simulink model "HAE"  (R2018a)
settings: Solver=ode4  StartTime=0  StopTime=2  MaxStep=1e-4  RelTol=1e-3
InitFcn:
  | close
  | clear
  | clc
  | Sc=128
  | f=60;
  | T=1/f;
  | Ts=1/(f*Sc);
  | Vr=6500
  | V_v=[1    0.4    1          0.6       1       0.6       1       0.75   0.95]
  | T_v=[0   20/f  70/f    200/f   300/f     330/f   400/f   500/f  10]
  | S_time=60/f*20.5
  | V_R=3;
  | Tf=3
  | T_lc=3
  | set_param('HAE/EMISOR-RECEPTOR/TCP_IP_RX1/ESCRITURA', 'Value','0')
  | set_param('HAE/EMISOR-RECEPTOR/TCP_IP_RX1/RETARDO', 'Value','0')
  | run script_client_1_inicio2.m
undefined symbols (not defined in the file or in its folder): D11, Delta, DiscIntNeverNeededParam, Int, Ip1
libraries: powerlib x68, simulink x12, powerlib_meascontrol x6, libreria_comunicaciones_cliente2 x2, libreria_medidores2 x1
(part 1 of 5)
settings Model: Creator=Mateo  LastModifiedBy=ana-n
settings CodeAppCC: StateflowObjectComments=on
settings SimscapeCC: SimscapeNormalizeSystem=off

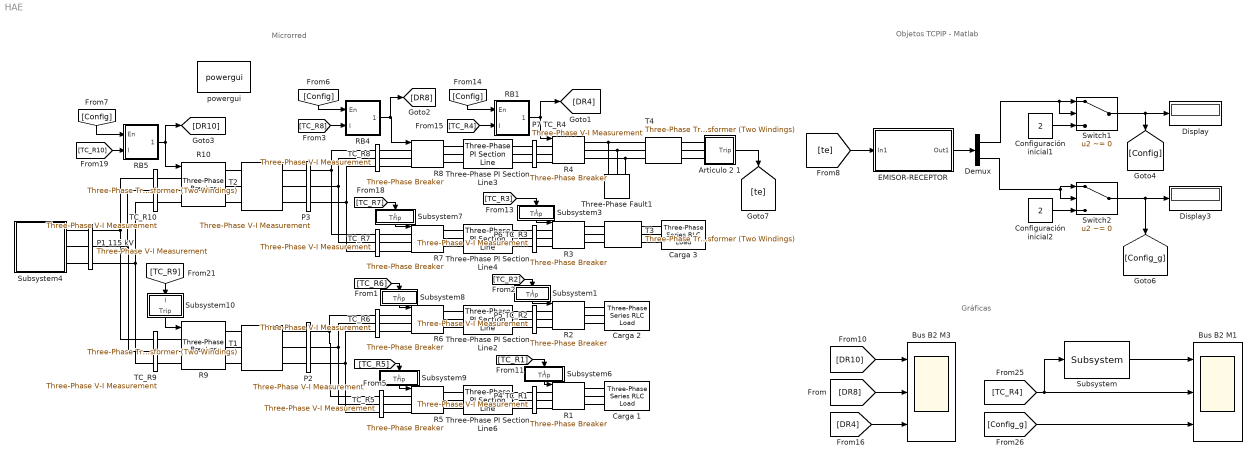
== system HAE ==
  note: Microrred
  note: Gráficas
  note: Objetos TCPIP - Matlab
  Articulo 2 1 : Subsystem  mask(Electric Arc Furnace Hyperbolic Model){Vp=200, Vat=50, m_Vat=0.01, RZs1=0.0528e-10, HZs1=1.4897e-10, RZc1=0.3366e-3, HZc1=0.01025e-3, Ci=190e3, Cd=39e3, Di_Dd=5e3, Constant_stages=[1 2 -15 0.5]}
      mask prompts: Vp "Peak Voltage"; RZs1 "RZs1 resistance Zs1"; HZs1 "HZs1 inductance Zs1"; RZc1 "RZc1 resistance Zc1"; HZc1 "HZc1 inductance Zc1"; Ci "Constant arc power Ci"; Cd "Constant arc power Cd"; Di_Dd "Constant arc current Did"; Constant_stages "Constants of each stage"
      mask help:
      | This model is based on the following documents:
      |
      | -Review on characteristic modeling of electric arc and its effects furnace
      | -Power system harmonics Computer modelling and analysis de Henrique Hacha y Manuel Madrigal
      | -Hornos de arco electrico Una vision desde la calidad de la potencia electrica
      |
      | This model recreates the time-varying, non-linear load behavior of the Electric Arc Furnaces.
      |
      | This model includes the possibility to add a time interval of different stages  of the tap-to-tap cycle as:
      |
      | -Furnance charging
      | -Melting.
      | -Refining
      | -De-slaging
      | -Furnace Turn-over
      |
      | The tap-to-tap cycle runs  through the simulation repeating the time intervals of the tap-to-tap cycle with different magnitudes in each cycle.
      |
      | The time of tap-to-tap cycle can be found in the book "Hornos de arco electrico Una vision desde la calidad de la potencia electrica" Table 2.3
      |
      | Additionaly considers the:
      | -Drilling period: Short period (between 3 to 4 minutes) using reduced voltages and powers. The material to be reduced, cause very irregular variations in the electric arc.
      | -Melting period: The electric arc is surrounded by melting scrap, which at this stage forms a more homogeneous material than in the drilling period. Full voltage and power is used in this process, lasting between 21 to 23 minutes. Typical values for medium power electric furnace are 610 V, 42 kA, 37 MW and PF 0.83.
      | -End of melting period and reheating: Uses lower voltage and higher current than in the melting period. It involves short arcs and last for about 5 minutes. Typical values in this process are 560 V, 45 kA, 34 MW and PF 0.78.
      |
      | To control the operation time of each of stages of the Tap-to-tap cycle, inside the model are differenciated as follows:
      | 1- Furnace charging
      | 2- Melting
      | 3- Refining and De-slaging
      | 4- Furnace turn-over
      mask Help:
      | This document implements the model of the Electric Arc Furnace (EAF) based on the following hyperbolic model.
      | 
      | V(I)=[V_T+(Ci,d)/(Di,d+abs(I))]signum(I)
      | 
      | Where I and V are the arc current and voltage of a given phase, respectively. In addition, V_T is the magnitude of the voltage threshold to which the voltage approaches as the current increases. This voltage is dependent on the arc length. Constants Ci,d and Di,d are corresponding to the arc power and arc current respectively, and regarding the sign of the derivative of the arc current, they can take different values. Since this equation is similar to the hyperbolic function, it is named hyperbolic model. There are different paths to increase or reduce the current.
      | 
      | The first describes the increasing current I(t), and the second the decreasing current (d).
      | 
      | Thus, constans Ci,d and Di,d are distinguised. The constants for the first path are Ci and Di and constans of the second path are Cd and Dd.
      | 
      | This model contemplates the possibility to change the time interval of the tap-to-tap cycle operation.
      | The so-called ultra-high-power furnaces, available since 1960, can have capacities of 50-150 tonnes, can have 12 melting cycles per day, opposed with 4 to 5 cycles achieved with previeous generations of furnaces.
      | 
      | Large variations are observed in the voltage and current measured during the drilling period, giving rise to a badly distorted v-i characteristic, which resembles more a transient operation than the steady-state operation. During the melting-down process the voltage and current waveforms are more regular but still the voltage is highly non-sinusoidal. At the end of the melting-down period, the voltage waveform becomes more sinusoidal and the v-i characteristic exhibits a high degree of linearity.
      | 
      | Rated Power of the transformer: 30 MVA
      | Transformer relation of the transformer 115/13.8 kV
      | Impedance of short circuit: 10,27% at 25 MVA
      | 
      | Rated short circuit power of the grid of the point of common coupling (115 kV).
      | Short circuit rated power 1653 MVA
      | Short circuit current 8300 A
      | 
      | Impedance of the transformer of the EAF. (Toshiba recommends)
      | Impedance Z% 5% - 6%
      | 
      | Maximun voltage at the secundary of the transformer.
      | Vmax=700 V
      | 
      | The time of the refining depends on the amount of tonns required (example of 38 Tonns). The EAF uses a 120 kWh/Tonn. Therefore,
      | 
      | E_required=(120kWh/Tonn)*(38 Tonn)=4560 kWh
      | 
      | - Complicated refining (more time required):
      | 
      | In consequence, the active required power is:
      | 
      | P_required=E_required/t_max_refining=4560 kWh*(60min/1h)*(1/40min)=6,8 MW
      | 
      | With the required active power is possible to compute the required aparent power (S) using the estimated power factor.
      | 
      | S_required=P_required/FP=6,8 MW/0,8 = 8,6 MVA
      | 
      | With a voltage of 380V the current is:
      | 
      | I=S_required/(sqrt(3)*V)=8,6MW/(sqrt(3)*380V)=13,1 kA
      | 
      | - Refining:
      | 
      | Refining stage: using the same EAF for the proces of refining, the estimated production takes t_max_refining = 20 min.
      | With this time the required power takes:
      | 
      | P_required=4560 kWh*(60min/1h)*(1/20min)=12,7 MW
      | S_required=12,7 MW/0,8 = 17 MVA
      | 
      | For a voltage of 500 V:
      | I=17MW/(sqrt(3)*500V)=19,6 kA
      | 
      | - Fusion stage
      | 
      | Fusion stage requires 400 kWh/T. Additionally the modeled EAF uses burners that use 466 kWh/min
      | 
      | E_required=(400kWh/Tonn)*(33 Tonn)=13200 kWh
      | t_fusion=E_required/Burning=13200 kWh/466 kWh/min=28 min
      | 
      | Wihtout burners, the Burning takes 400 kWh/min
      | 
      | t_fusion=E_required/Burning=13200 kWh/400 kWh/min=33 min
      | 
      | - Time of charging and turn-over
      | 
      | The time of the charging to transport the scrapping and how to fill the furnace. Estimating 4 loads to charge the furnace in 3 minutes it takes.
      | 
      | t_charging=(# charging)*(time of charging)=4*3 min=12 min
      | Time of turn-over: 10 minutes.
      | 
      | Therefore, consider a time interval for the tap-to-tap cycle of 60 min - 85 min, as follows:
      | 
      | -Furnace Charging: 12 minutes
      | -Melting: 28 minutes
      | -Refining and De-slaging: 20 minutes
      | -Furnace turn-over: 10 minutes
      | 
      | Considering 70 cycles as a hole tap-to-tap cycle, the following time interval is considered:
      | 
      | -Furnace Charging: 12 cycles
      | -Melting: 28 cycles
      | -Refining and De-slaging: 20 cycles
      | -Furnace turn-over: 10 cycles
      mask Display: disp('HAE');
  Bus B2 M1 : Scope  NumInputPorts=3
  Bus B2 M3 : Scope  NumInputPorts=3
  Carga 1 : powerlib/Elements/Three-Phase Series RLC Load  LConnTagsString=A|B|C  Configuration=Y (grounded)  NominalVoltage=13.8e3  Vabc=[1e3 1e3 1e3]  Vabcp=[1e3 1e3 1e3]  NominalFrequency=60  UnbalancedPower=off  ActivePower=35e5  InductivePower=3e5  CapacitivePower=0  Pabc=[10e3 9e3 11e3]  QLabc=[100 90 110]  QCabc=[100 90 110]  Pabcp=[10e3 9e3 11e3]  QLabcp=[100 90 110]  QCabcp=[100 90 110]  Measurements=None  LoadType=constant PQ
  Carga 2 : powerlib/Elements/Three-Phase Series RLC Load  LConnTagsString=A|B|C  Configuration=Y (grounded)  NominalVoltage=13.8e3  Vabc=[1e3 1e3 1e3]  Vabcp=[1e3 1e3 1e3]  NominalFrequency=60  UnbalancedPower=off  ActivePower=35e5  InductivePower=3e5  CapacitivePower=0  Pabc=[10e3 9e3 11e3]  QLabc=[100 90 110]  QCabc=[100 90 110]  Pabcp=[10e3 9e3 11e3]  QLabcp=[100 90 110]  QCabcp=[100 90 110]  Measurements=None  LoadType=constant PQ
  Carga 3 : powerlib/Elements/Three-Phase Series RLC Load  LConnTagsString=A|B|C  Configuration=Y (grounded)  NominalVoltage=0.480e3  Vabc=[1e3 1e3 1e3]  Vabcp=[1e3 1e3 1e3]  NominalFrequency=60  UnbalancedPower=off  ActivePower=6e6  InductivePower=0.5e6  CapacitivePower=0  Pabc=[10e3 9e3 11e3]  QLabc=[100 90 110]  QCabc=[100 90 110]  Pabcp=[10e3 9e3 11e3]  QLabcp=[100 90 110]  QCabcp=[100 90 110]  Measurements=None  LoadType=constant PQ
  Configuración inicial1 : Constant  Value=2
  Configuración inicial2 : Constant  Value=2
  Demux : Demux  Outputs=2
  Display : Display
  Display3 : Display
  EMISOR-RECEPTOR : Subsystem
      mask Display: disp("Emisor-Receptor")
  P1 115 kV : powerlib/Measurements/Three-Phase V-I Measurement  VoltageMeasurement=phase-to-ground  SetLabelV=on  LabelV=V_B_P1  Vpu=off  VpuLL=off  CurrentMeasurement=yes  SetLabelI=on  LabelI=I_B_P1  Ipu=off  Pbase=100e6  Vbase=500e3  OutputType=Complex  PhasorSimulation=off  PSBequivalent=0
  P2 : powerlib/Measurements/Three-Phase V-I Measurement  VoltageMeasurement=phase-to-ground  SetLabelV=on  LabelV=V_F_F2  Vpu=off  VpuLL=off  CurrentMeasurement=yes  SetLabelI=on  LabelI=I_F_F2  Ipu=off  Pbase=100e6  Vbase=500e3  OutputType=Complex  PhasorSimulation=off  PSBequivalent=0
  P3 : powerlib/Measurements/Three-Phase V-I Measurement  VoltageMeasurement=phase-to-ground  SetLabelV=on  LabelV=V_F_F3  Vpu=off  VpuLL=off  CurrentMeasurement=yes  SetLabelI=on  LabelI=I_F_F3  Ipu=off  Pbase=100e6  Vbase=500e3  OutputType=Complex  PhasorSimulation=off  PSBequivalent=0
  P4 TC_R1 : powerlib/Measurements/Three-Phase V-I Measurement  VoltageMeasurement=phase-to-ground  SetLabelV=on  LabelV=V_RM_1  Vpu=off  VpuLL=off  CurrentMeasurement=yes  SetLabelI=on  LabelI=TC_R1  Ipu=off  Pbase=100e6  Vbase=500e3  OutputType=Complex  PhasorSimulation=off  PSBequivalent=0
  P5 TC_R2 : powerlib/Measurements/Three-Phase V-I Measurement  VoltageMeasurement=phase-to-ground  SetLabelV=on  LabelV=V_F_RM_2  Vpu=off  VpuLL=off  CurrentMeasurement=yes  SetLabelI=on  LabelI=TC_R2  Ipu=off  Pbase=100e6  Vbase=500e3  OutputType=Complex  PhasorSimulation=off  PSBequivalent=0
  P6 TC_R3 : powerlib/Measurements/Three-Phase V-I Measurement  VoltageMeasurement=phase-to-ground  SetLabelV=on  LabelV=V_HV_L3  Vpu=off  VpuLL=off  CurrentMeasurement=yes  SetLabelI=on  LabelI=TC_R3  Ipu=off  Pbase=100e6  Vbase=500e3  OutputType=Complex  PhasorSimulation=off  PSBequivalent=0
  P7 TC_R4 : powerlib/Measurements/Three-Phase V-I Measurement  VoltageMeasurement=phase-to-ground  SetLabelV=on  LabelV=V_HV_7  Vpu=off  VpuLL=off  CurrentMeasurement=yes  SetLabelI=on  LabelI=TC_R4  Ipu=off  Pbase=100e6  Vbase=500e3  OutputType=Complex  PhasorSimulation=off  PSBequivalent=0
  R1 : powerlib/Elements/Three-Phase Breaker  InitialState=closed  SwitchA=on  SwitchB=on  SwitchC=on  SwitchTimes=[5]  External=on  BreakerResistance=0.001  SnubberResistance=1e6  SnubberCapacitance=inf  Measurements=None
      link override Breaker A: Measurements=None
      link override Breaker B: Measurements=None
      link override Breaker C: Measurements=None
  R10 : powerlib/Elements/Three-Phase Breaker  InitialState=closed  SwitchA=on  SwitchB=on  SwitchC=on  SwitchTimes=[5]  External=on  BreakerResistance=0.001  SnubberResistance=1e6  SnubberCapacitance=inf  Measurements=None
      link override Breaker A: Measurements=None
      link override Breaker B: Measurements=None
      link override Breaker C: Measurements=None
  R2 : powerlib/Elements/Three-Phase Breaker  InitialState=closed  SwitchA=on  SwitchB=on  SwitchC=on  SwitchTimes=[5]  External=on  BreakerResistance=0.001  SnubberResistance=1e6  SnubberCapacitance=inf  Measurements=None
      link override Breaker A: Measurements=None
      link override Breaker B: Measurements=None
      link override Breaker C: Measurements=None
  R3 : powerlib/Elements/Three-Phase Breaker  InitialState=closed  SwitchA=on  SwitchB=on  SwitchC=on  SwitchTimes=[5]  External=on  BreakerResistance=0.001  SnubberResistance=1e6  SnubberCapacitance=inf  Measurements=None
      link override Breaker A: Measurements=None
      link override Breaker B: Measurements=None
      link override Breaker C: Measurements=None
  R4 : powerlib/Elements/Three-Phase Breaker  InitialState=closed  SwitchA=on  SwitchB=on  SwitchC=on  SwitchTimes=[20]  External=on  BreakerResistance=0.001  SnubberResistance=1e6  SnubberCapacitance=inf  Measurements=None
      link override Breaker A: Measurements=None
      link override Breaker B: Measurements=None
      link override Breaker C: Measurements=None
  R5 : powerlib/Elements/Three-Phase Breaker  InitialState=closed  SwitchA=on  SwitchB=on  SwitchC=on  SwitchTimes=[5]  External=on  BreakerResistance=0.001  SnubberResistance=1e6  SnubberCapacitance=inf  Measurements=None
      link override Breaker A: Measurements=None
      link override Breaker B: Measurements=None
      link override Breaker C: Measurements=None
  R6 : powerlib/Elements/Three-Phase Breaker  InitialState=closed  SwitchA=on  SwitchB=on  SwitchC=on  SwitchTimes=[5]  External=on  BreakerResistance=0.001  SnubberResistance=1e6  SnubberCapacitance=inf  Measurements=None
      link override Breaker A: Measurements=None
      link override Breaker B: Measurements=None
      link override Breaker C: Measurements=None
  R7 : powerlib/Elements/Three-Phase Breaker  InitialState=closed  SwitchA=on  SwitchB=on  SwitchC=on  SwitchTimes=[5]  External=on  BreakerResistance=0.001  SnubberResistance=1e6  SnubberCapacitance=inf  Measurements=None
      link override Breaker A: Measurements=None
      link override Breaker B: Measurements=None
      link override Breaker C: Measurements=None
  R8 : powerlib/Elements/Three-Phase Breaker  InitialState=closed  SwitchA=on  SwitchB=on  SwitchC=on  SwitchTimes=[20]  External=on  BreakerResistance=0.001  SnubberResistance=1e6  SnubberCapacitance=inf  Measurements=None
      link override Breaker A: Measurements=None
      link override Breaker B: Measurements=None
      link override Breaker C: Measurements=None
  R9 : powerlib/Elements/Three-Phase Breaker  InitialState=closed  SwitchA=on  SwitchB=on  SwitchC=on  SwitchTimes=[5]  External=on  BreakerResistance=0.001  SnubberResistance=1e6  SnubberCapacitance=inf  Measurements=None
      link override Breaker A: Measurements=None
      link override Breaker B: Measurements=None
      link override Breaker C: Measurements=None
  RB1 : Subsystem  mask(Proteccion de Sobrecorriente multitopologia){menu=3, TCpopup1=IEC Standard Inverse, k1=0.14, alpha1=0.02, B1=0, PS1=0.10, TMS1=0.5, Tins1=0.015, Esc1=10, TCpopup2=IEC Standard Inverse, k2=0.14, alpha2=0.02, B2=0, PS2=1, TMS2=0.060, Tins2=0.09, Esc2=5, TCpopup3=IEC Standard Inverse, k3=0.14, alpha3=0.02, B3=0, PS3=0.6267, TMS3=0.100, Tins3=0.05, Esc3=4, Vp=1200, Vs=5, F=60}
      mask prompts: menu "Numero de Topologias"; TCpopup1 "Caracteristica de Disparo"; k1 "k"; alpha1 "alpha"; B1 "B"; PS1 "Seteo disparo(PS)/Seteo inferior(I>)"; TMS1 "Multiplicador de Tiempo"; Tins1 "Tins"; Esc1 "Escala"; TCpopup2 "Caracteristica de Disparo"; k2 "k"; alpha2 "alpha"; B2 "B"; PS2 "Seteo disparo(PS)/Seteo inferior(I>)"; TMS2 "Multiplicador de tiempo"; Tins2 "Tins"; Esc2 "Escala"; TCpopup3 "Caracteristica de Disparo"; k3 "k"; alpha3 "alpha"; B3 "B"; PS3 "Seteo disparo(PS)/Seteo inferior(I>)"; TMS3 "Multiplicador de Tiempo"; Tins3 "Tins"; Esc3 "Escala"; Vp "Primario CT"; Vs "Secundario CT"; F "Frecuencia"
      mask help: Proteccion de Sobrecorriente con tres topologias internas controladas por una señal de control externa.
      mask init:
      | warning('off','Simulink:Masking:Invalid_Visible_Flag')
      mask TypeOptions menu: 1 | 2 | 3
      mask Callback menu:
      | h = getSimulinkBlockHandle(gcb);
      | menu1 = get_param(h,'menu');
      | if strcmp(menu1,num2str(1))
      |     set_param(h,'MaskVisibilities',{'on',...
      |         'on','on','on','on','on','on','on','on',...%proteccion 1 activa
      |         'off','off','off','off','off','off','off','off',...%proteccion 2 desactivada
      |         'off','off','off','off','off','off','off','off',...%proteccion 3 desactivada
      |         'on','on','on'});%Otros parametros activados
      |     Int=1;
      | elseif strcmp(menu1,num2str(2))
      |  set_param(h,'MaskVisibilities',{'on',...
      |         'on','on','on','on','on','on','on','on',...%proteccion 1 activa
      |         'on','on','on','on','on','on','on','on',...%proteccion 2 activa
      |         'off','off','off','off','off','off','off','off',...%proteccion 3 desactivada
      |         'on','on','on'});%Otros parametros activados
      |     Int=2;
      | else
      | set_param(h,'MaskVisibilities',{'on',...
      |         'on','on','on','on','on','on','on','on',...%proteccion 1 activa
      |         'on','on','on','on','on','on','on','on',...%proteccion 2 activa
      |         'on','on','on','on','on','on','on','on',...%proteccion 3 desactivada
      |         'on','on','on'});%Otros parametros activados
      |     Int=3;
      | end
      mask TypeOptions TCpopup1: IEC Standard Inverse | IEC Very Inverse | IEC Long Time Inverse | IEC Extremely Inverse | IEC Ultra Inverse | IEEE Moderately Inverse | IEEE Very Inverse | IEEE Extremely Inverse
      mask Callback TCpopup1:
      | switch(get_param(gcb,'TCpopup1'))
      |     case 'IEC Standard Inverse'
      |         set_param(gcb,'k1','0.14');
      |         set_param(gcb,'alpha1','0.02');
      |         set_param(gcb,'B1','0');
      |     case 'IEC Very Inverse'
      |         set_param(gcb,'k1','13.5');
      |         set_param(gcb,'alpha1','1');
      |         set_param(gcb,'B1','0');
      |     case 'IEC Long Time Inverse'
      |         set_param(gcb,'k1','120');
      |         set_param(gcb,'alpha1','1');
      |         set_param(gcb,'B1','0');
      |     case 'IEC Extremely Inverse'
      |         set_param(gcb,'k1','80');
      |         set_param(gcb,'alpha1','2');
      |         set_param(gcb,'B1','0');
      |     case 'IEC Ultra Inverse'
      |         set_param(gcb,'k1','315.2');
      |         set_param(gcb,'alpha1','2.5');
      |         set_param(gcb,'B1','0');
      |     case 'IEEE Moderately Inverse'
      |         set_param(gcb,'k1','0.0515');
      |         set_param(gcb,'alpha1','0.02');
      |         set_param(gcb,'B1','0.114');
      |     case 'IEEE Very Inverse'
      |         set_param(gcb,'k1','19.61');
      |         set_param(gcb,'alpha1','2');
      |         set_param(gcb,'B1','0.491');
      |     case 'IEEE Extremely Inverse'
      |         set_param(gcb,'k1','28.2');
      |         set_param(gcb,'alpha1','2');
      |         set_param(gcb,'B1','0.1217');
      | end
      | % Plotting IDMT Curve
      | clf('reset')
      | TMS = str2num(get_param(gcb,'TMS1'));
      | Vp = str2num(get_param(gcb,'Vp'));
      | PS=str2num(get_param(gcb,'PS1'));
      | k = str2num(get_param(gcb,'k1'));
      | alpha = str2num(get_param(gcb,'alpha1'));
      | B = str2num(get_param(gcb,'B1'));
      | Esc = str2num(get_param(gcb,'Esc1'));
      | Tins = str2num(get_param(gcb,'Tins1'));
      | I = [1.1:0.1:Esc];
      | I1=[Esc,Esc:0.1:30];
      | y=((k./((I.^alpha)-1))+B)*TMS;
      | Tin=[((k./((Esc.^alpha)-1))+B)*TMS,ones(1,length(I1)-1)*Tins];
      | loglog(I,y,'b');
      | hold on
      | loglog(I1,Tin,'b');
      | set(gcf, 'Position', [200 150 300 500]);
      | switch(get_param(gcb,'TCpopup1'))
      |     case 'IEC Standard Inverse'
      |         title('IEC Standard Inverse');
      |     case 'IEC Very Inverse'
      |         title('IEC Very Inverse');
      |     case 'IEC Long Time Inverse'
      |         title('IEC Long Time Inverse');
      |     case 'IEC Extremely Inverse'
      |         title('IEC Extremely Inverse');
      |      case 'IEC Ultra Inverse'
      |         title('IEC Ultra Inverse');
      |     case 'IEEE Moderately Inverse'
      |         title('IEEE Moderately Inverse');
      |     case 'IEEE Very Inverse'
      |         title('IEEE Very Inverse');
      |     case 'IEEE Extremely Inverse'
      |         title('IEEE Extremely Inverse');
      | end
      | ymax=10^ceil(log10(max(y)));
      | set(gca, 'XTick',[1:10 20]);
      | set(gca, 'YTick',[0 ymax/1000 ymax/500 ymax/200 ymax/100 ymax/50 ymax/20 ymax/10 ymax/5 ymax/2 ymax]);
      | xlim([0.9 30]);
      | ylim([0.01 ymax]);
      | xlabel(['Corriente multiplicada por Ipick-up(' num2str(PS*Vp) 'A)']);
      | ylabel('Tiempo de Operacion (Seg)');
      | grid on;
      | set(gca, 'color',[0.9608 0.9608 0.937]);
      | set(gca, 'gridcolor',[0 0.6902 0.3137]);
      mask Callback PS1:
      | % Plotting IDMT Curve
      | clf('reset')
      | TMS = str2num(get_param(gcb,'TMS1'));
      | Vp = str2num(get_param(gcb,'Vp'));
      | PS=str2num(get_param(gcb,'PS1'));
      | k = str2num(get_param(gcb,'k1'));
      | alpha = str2num(get_param(gcb,'alpha1'));
      | B = str2num(get_param(gcb,'B1'));
      | Esc = str2num(get_param(gcb,'Esc1'));
      | Tins = str2num(get_param(gcb,'Tins1'));
      | I = [1.1:0.1:Esc];
      | I1=[Esc,Esc:0.1:30];
      | y=((k./((I.^alpha)-1))+B)*TMS;
      | Tin=[((k./((Esc.^alpha)-1))+B)*TMS,ones(1,length(I1)-1)*Tins];
      | loglog(I,y,'b');
      | hold on
      | loglog(I1,Tin,'b');
      | set(gcf, 'Position', [200 150 300 500]);
      | switch(get_param(gcb,'TCpopup1'))
      |     case 'IEC Standard Inverse'
      |         title('IEC Standard Inverse');
      |     case 'IEC Very Inverse'
      |         title('IEC Very Inverse');
      |     case 'IEC Long Time Inverse'
      |         title('IEC Long Time Inverse');
      |     case 'IEC Extremely Inverse'
      |         title('IEC Extremely Inverse');
      |      case 'IEC Ultra Inverse'
      |         title('IEC Ultra Inverse');
      |     case 'IEEE Moderately Inverse'
      |         title('IEEE Moderately Inverse');
      |     case 'IEEE Very Inverse'
      |         title('IEEE Very Inverse');
      |     case 'IEEE Extremely Inverse'
      |         title('IEEE Extremely Inverse');
      | end
      | ymax=10^ceil(log10(max(y)));
      | set(gca, 'XTick',[1:10 20]);
      | set(gca, 'YTick',[0 ymax/1000 ymax/500 ymax/200 ymax/100 ymax/50 ymax/20 ymax/10 ymax/5 ymax/2 ymax]);
      | xlim([0.9 30]);
      | ylim([0.01 ymax]);
      | xlabel(['Corriente multiplicada por Ipick-up(' num2str(PS*Vp) 'A)']);
      | ylabel('Tiempo de Operacion (Seg)');
      | grid on;
      | set(gca, 'color',[0.9608 0.9608 0.937]);
      | set(gca, 'gridcolor',[0 0.6902 0.3137]);
      mask Callback TMS1:
      | % Plotting IDMT Curve
      | clf('reset')
      | TMS = str2num(get_param(gcb,'TMS1'));
      | Vp = str2num(get_param(gcb,'Vp'));
      | PS=str2num(get_param(gcb,'PS1'));
      | k = str2num(get_param(gcb,'k1'));
      | alpha = str2num(get_param(gcb,'alpha1'));
      | B = str2num(get_param(gcb,'B1'));
      | Esc = str2num(get_param(gcb,'Esc1'));
      | Tins = str2num(get_param(gcb,'Tins1'));
      | I = [1.1:0.1:Esc];
      | I1=[Esc,Esc:0.1:30];
      | y=((k./((I.^alpha)-1))+B)*TMS;
      | Tin=[((k./((Esc.^alpha)-1))+B)*TMS,ones(1,length(I1)-1)*Tins];
      | loglog(I,y,'b');
      | hold on
      | loglog(I1,Tin,'b');
      | set(gcf, 'Position', [200 150 300 500]);
      | switch(get_param(gcb,'TCpopup1'))
      |     case 'IEC Standard Inverse'
      |         title('IEC Standard Inverse');
      |     case 'IEC Very Inverse'
      |         title('IEC Very Inverse');
      |     case 'IEC Long Time Inverse'
      |         title('IEC Long Time Inverse');
      |     case 'IEC Extremely Inverse'
      |         title('IEC Extremely Inverse');
      |      case 'IEC Ultra Inverse'
      |         title('IEC Ultra Inverse');
      |     case 'IEEE Moderately Inverse'
      |         title('IEEE Moderately Inverse');
      |     case 'IEEE Very Inverse'
      |         title('IEEE Very Inverse');
      |     case 'IEEE Extremely Inverse'
      |         title('IEEE Extremely Inverse');
      | end
      | ymax=10^ceil(log10(max(y)));
      | set(gca, 'XTick',[1:10 20]);
      | set(gca, 'YTick',[0 ymax/1000 ymax/500 ymax/200 ymax/100 ymax/50 ymax/20 ymax/10 ymax/5 ymax/2 ymax]);
      | xlim([0.9 30]);
      | ylim([0.01 ymax]);
      | xlabel(['Corriente multiplicada por Ipick-up(' num2str(PS*Vp) 'A)']);
      | ylabel('Tiempo de Operacion (Seg)');
      | grid on;
      | set(gca, 'color',[0.9608 0.9608 0.937]);
      | set(gca, 'gridcolor',[0 0.6902 0.3137]);
      mask Callback Tins1:
      | % Plotting IDMT Curve
      | clf('reset')
      | TMS = str2num(get_param(gcb,'TMS1'));
      | Vp = str2num(get_param(gcb,'Vp'));
      | PS=str2num(get_param(gcb,'PS1'));
      | k = str2num(get_param(gcb,'k1'));
      | alpha = str2num(get_param(gcb,'alpha1'));
      | B = str2num(get_param(gcb,'B1'));
      | Esc = str2num(get_param(gcb,'Esc1'));
      | Tins = str2num(get_param(gcb,'Tins1'));
      | I = [1.1:0.1:Esc];
      | I1=[Esc,Esc:0.1:30];
      | y=((k./((I.^alpha)-1))+B)*TMS;
      | Tin=[((k./((Esc.^alpha)-1))+B)*TMS,ones(1,length(I1)-1)*Tins];
      | loglog(I,y,'b');
      | hold on
      | loglog(I1,Tin,'b');
      | set(gcf, 'Position', [200 150 300 500]);
      | switch(get_param(gcb,'TCpopup1'))
      |     case 'IEC Standard Inverse'
      |         title('IEC Standard Inverse');
      |     case 'IEC Very Inverse'
      |         title('IEC Very Inverse');
      |     case 'IEC Long Time Inverse'
      |         title('IEC Long Time Inverse');
      |     case 'IEC Extremely Inverse'
      |         title('IEC Extremely Inverse');
      |      case 'IEC Ultra Inverse'
      |         title('IEC Ultra Inverse');
      |     case 'IEEE Moderately Inverse'
      |         title('IEEE Moderately Inverse');
      |     case 'IEEE Very Inverse'
      |         title('IEEE Very Inverse');
      |     case 'IEEE Extremely Inverse'
      |         title('IEEE Extremely Inverse');
      | end
      | ymax=10^ceil(log10(max(y)));
      | set(gca, 'XTick',[1:10 20]);
      | set(gca, 'YTick',[0 ymax/1000 ymax/500 ymax/200 ymax/100 ymax/50 ymax/20 ymax/10 ymax/5 ymax/2 ymax]);
      | xlim([0.9 30]);
      | ylim([0.01 ymax]);
      | xlabel(['Corriente multiplicada por Ipick-up(' num2str(PS*Vp) 'A)']);
      | ylabel('Tiempo de Operacion (Seg)');
      | grid on;
      | set(gca, 'color',[0.9608 0.9608 0.937]);
      | set(gca, 'gridcolor',[0 0.6902 0.3137]);
      mask Callback Esc1:
      | % Plotting IDMT Curve
      | clf('reset')
      | TMS = str2num(get_param(gcb,'TMS1'));
      | Vp = str2num(get_param(gcb,'Vp'));
      | PS=str2num(get_param(gcb,'PS1'));
      | k = str2num(get_param(gcb,'k1'));
      | alpha = str2num(get_param(gcb,'alpha1'));
      | B = str2num(get_param(gcb,'B1'));
      | Esc = str2num(get_param(gcb,'Esc1'));
      | Tins = str2num(get_param(gcb,'Tins1'));
      | I = [1.1:0.1:Esc];
      | I1=[Esc,Esc:0.1:30];
      | y=((k./((I.^alpha)-1))+B)*TMS;
      | Tin=[((k./((Esc.^alpha)-1))+B)*TMS,ones(1,length(I1)-1)*Tins];
      | loglog(I,y,'b');
      | hold on
      | loglog(I1,Tin,'b');
      | set(gcf, 'Position', [200 150 300 500]);
      | switch(get_param(gcb,'TCpopup1'))
      |     case 'IEC Standard Inverse'
      |         title('IEC Standard Inverse');
      |     case 'IEC Very Inverse'
      |         title('IEC Very Inverse');
      |     case 'IEC Long Time Inverse'
      |         title('IEC Long Time Inverse');
      |     case 'IEC Extremely Inverse'
      |         title('IEC Extremely Inverse');
      |      case 'IEC Ultra Inverse'
      |         title('IEC Ultra Inverse');
      |     case 'IEEE Moderately Inverse'
      |         title('IEEE Moderately Inverse');
      |     case 'IEEE Very Inverse'
      |         title('IEEE Very Inverse');
      |     case 'IEEE Extremely Inverse'
      |         title('IEEE Extremely Inverse');
      | end
      | ymax=10^ceil(log10(max(y)));
      | set(gca, 'XTick',[1:10 20]);
      | set(gca, 'YTick',[0 ymax/1000 ymax/500 ymax/200 ymax/100 ymax/50 ymax/20 ymax/10 ymax/5 ymax/2 ymax]);
      | xlim([0.9 30]);
      | ylim([0.01 ymax]);
      | xlabel(['Corriente multiplicada por Ipick-up(' num2str(PS*Vp) 'A)']);
      | ylabel('Tiempo de Operacion (Seg)');
      | grid on;
      | set(gca, 'color',[0.9608 0.9608 0.937]);
      | set(gca, 'gridcolor',[0 0.6902 0.3137]);
      mask TypeOptions TCpopup2: IEC Standard Inverse | IEC Very Inverse | IEC Long Time Inverse | IEC Extremely Inverse | IEC Ultra Inverse | IEEE Moderately Inverse | IEEE Very Inverse | IEEE Extremely Inverse
      mask Callback TCpopup2:
      | switch(get_param(gcb,'TCpopup2'))
      |     case 'IEC Standard Inverse'
      |         set_param(gcb,'k2','0.14');
      |         set_param(gcb,'alpha2','0.02');
      |         set_param(gcb,'B2','0');
      |     case 'IEC Very Inverse'
      |         set_param(gcb,'k2','13.5');
      |         set_param(gcb,'alpha2','1');
      |         set_param(gcb,'B2','0');
      |     case 'IEC Long Time Inverse'
      |         set_param(gcb,'k2','120');
      |         set_param(gcb,'alpha2','1');
      |         set_param(gcb,'B2','0');
      |     case 'IEC Extremely Inverse'
      |         set_param(gcb,'k2','80');
      |         set_param(gcb,'alpha2','2');
      |         set_param(gcb,'B2','0');
      |     case 'IEC Ultra Inverse'
      |         set_param(gcb,'k2','315.2');
      |         set_param(gcb,'alpha2','2.5');
      |         set_param(gcb,'B2','0');
      |     case 'IEEE Moderately Inverse'
      |         set_param(gcb,'k2','0.0515');
      |         set_param(gcb,'alpha2','0.02');
      |         set_param(gcb,'B2','0.114');
      |     case 'IEEE Very Inverse'
      |         set_param(gcb,'k2','19.61');
      |         set_param(gcb,'alpha2','2');
      |         set_param(gcb,'B2','0.491');
      |     case 'IEEE Extremely Inverse'
      |         set_param(gcb,'k2','28.2');
      |         set_param(gcb,'alpha2','2');
      |         set_param(gcb,'B2','0.1217');
      | end
      | % Plotting IDMT Curve
      | clf('reset')
      | TMS = str2num(get_param(gcb,'TMS2'));
      | Vp = str2num(get_param(gcb,'Vp'));
      | PS=str2num(get_param(gcb,'PS2'));
      | k = str2num(get_param(gcb,'k2'));
      | alpha = str2num(get_param(gcb,'alpha2'));
      | B = str2num(get_param(gcb,'B2'));
      | Esc = str2num(get_param(gcb,'Esc2'));
      | Tins = str2num(get_param(gcb,'Tins2'));
      | I = [1.1:0.1:Esc];
      | I1=[Esc,Esc:0.1:30];
      | y=((k./((I.^alpha)-1))+B)*TMS;
      | Tin=[((k./((Esc.^alpha)-1))+B)*TMS,ones(1,length(I1)-1)*Tins];
      | loglog(I,y,'r');
      | hold on
      | loglog(I1,Tin,'r');
      | set(gcf, 'Position', [200 150 300 500]);
      | switch(get_param(gcb,'TCpopup2'))
      |     case 'IEC Standard Inverse'
      |         title('IEC Standard Inverse');
      |     case 'IEC Very Inverse'
      |         title('IEC Very Inverse');
      |     case 'IEC Long Time Inverse'
      |         title('IEC Long Time Inverse');
      |     case 'IEC Extremely Inverse'
      |         title('IEC Extremely Inverse');
      |      case 'IEC Ultra Inverse'
      |         title('IEC Ultra Inverse');
      |     case 'IEEE Moderately Inverse'
      |         title('IEEE Moderately Inverse');
      |     case 'IEEE Very Inverse'
      |         title('IEEE Very Inverse');
      |     case 'IEEE Extremely Inverse'
      |         title('IEEE Extremely Inverse');
      | end
      | ymax=10^ceil(log10(max(y)));
      | set(gca, 'XTick',[1:10 20]);
      | set(gca, 'YTick',[0 ymax/1000 ymax/500 ymax/200 ymax/100 ymax/50 ymax/20 ymax/10 ymax/5 ymax/2 ymax]);
      | xlim([0.9 30]);
      | ylim([0.01 ymax]);
      | xlabel(['Corriente multiplicada por Ipick-up(' num2str(PS*Vp) 'A)']);
      | ylabel('Tiempo de Operacion (Seg)');
      | grid on;
      | set(gca, 'color',[0.9608 0.9608 0.937]);
      | set(gca, 'gridcolor',[0 0.6902 0.3137]);
      mask Callback PS2:
      | % Plotting IDMT Curve
      | clf('reset')
      | TMS = str2num(get_param(gcb,'TMS2'));
      | Vp = str2num(get_param(gcb,'Vp'));
      | PS=str2num(get_param(gcb,'PS2'));
      | k = str2num(get_param(gcb,'k2'));
      | alpha = str2num(get_param(gcb,'alpha2'));
      | B = str2num(get_param(gcb,'B2'));
      | Esc = str2num(get_param(gcb,'Esc2'));
      | Tins = str2num(get_param(gcb,'Tins2'));
      | I = [1.1:0.1:Esc];
      | I1=[Esc,Esc:0.1:30];
      | y=((k./((I.^alpha)-1))+B)*TMS;
      | Tin=[((k./((Esc.^alpha)-1))+B)*TMS,ones(1,length(I1)-1)*Tins];
      | loglog(I,y,'r');
      | hold on
      | loglog(I1,Tin,'r');
      | set(gcf, 'Position', [200 150 300 500]);
      | switch(get_param(gcb,'TCpopup2'))
      |     case 'IEC Standard Inverse'
      |         title('IEC Standard Inverse');
      |     case 'IEC Very Inverse'
      |         title('IEC Very Inverse');
      |     case 'IEC Long Time Inverse'
      |         title('IEC Long Time Inverse');
      |     case 'IEC Extremely Inverse'
      |         title('IEC Extremely Inverse');
      |      case 'IEC Ultra Inverse'
      |         title('IEC Ultra Inverse');
      |     case 'IEEE Moderately Inverse'
      |         title('IEEE Moderately Inverse');
      |     case 'IEEE Very Inverse'
      |         title('IEEE Very Inverse');
      |     case 'IEEE Extremely Inverse'
      |         title('IEEE Extremely Inverse');
      | end
      | ymax=10^ceil(log10(max(y)));
      | set(gca, 'XTick',[1:10 20]);
      | set(gca, 'YTick',[0 ymax/1000 ymax/500 ymax/200 ymax/100 ymax/50 ymax/20 ymax/10 ymax/5 ymax/2 ymax]);
      | xlim([0.9 30]);
      | ylim([0.01 ymax]);
      | xlabel(['Corriente multiplicada por Ipick-up(' num2str(PS*Vp) 'A)']);
      | ylabel('Tiempo de Operacion (Seg)');
      | grid on;
      | set(gca, 'color',[0.9608 0.9608 0.937]);
      | set(gca, 'gridcolor',[0 0.6902 0.3137]);
      mask Callback TMS2:
      | % Plotting IDMT Curve
      | clf('reset')
      | TMS = str2num(get_param(gcb,'TMS2'));
      | Vp = str2num(get_param(gcb,'Vp'));
      | PS=str2num(get_param(gcb,'PS2'));
      | k = str2num(get_param(gcb,'k2'));
      | alpha = str2num(get_param(gcb,'alpha2'));
      | B = str2num(get_param(gcb,'B2'));
      | Esc = str2num(get_param(gcb,'Esc2'));
      | Tins = str2num(get_param(gcb,'Tins2'));
      | I = [1.1:0.1:Esc];
      | I1=[Esc,Esc:0.1:30];
      | y=((k./((I.^alpha)-1))+B)*TMS;
      | Tin=[((k./((Esc.^alpha)-1))+B)*TMS,ones(1,length(I1)-1)*Tins];
      | loglog(I,y,'r');
      | hold on
      | loglog(I1,Tin,'r');
      | set(gcf, 'Position', [200 150 300 500]);
      | switch(get_param(gcb,'TCpopup2'))
      |     case 'IEC Standard Inverse'
      |         title('IEC Standard Inverse');
      |     case 'IEC Very Inverse'
      |         title('IEC Very Inverse');
      |     case 'IEC Long Time Inverse'
      |         title('IEC Long Time Inverse');
      |     case 'IEC Extremely Inverse'
      |         title('IEC Extremely Inverse');
      |      case 'IEC Ultra Inverse'
      |         title('IEC Ultra Inverse');
      |     case 'IEEE Moderately Inverse'
      |         title('IEEE Moderately Inverse');
      |     case 'IEEE Very Inverse'
      |         title('IEEE Very Inverse');
      |     case 'IEEE Extremely Inverse'
      |         title('IEEE Extremely Inverse');
      | end
      | ymax=10^ceil(log10(max(y)));
      | set(gca, 'XTick',[1:10 20]);
      | set(gca, 'YTick',[0 ymax/1000 ymax/500 ymax/200 ymax/100 ymax/50 ymax/20 ymax/10 ymax/5 ymax/2 ymax]);
      | xlim([0.9 30]);
      | ylim([0.01 ymax]);
      | xlabel(['Corriente multiplicada por Ipick-up(' num2str(PS*Vp) 'A)']);
      | ylabel('Tiempo de Operacion (Seg)');
      | grid on;
      | set(gca, 'color',[0.9608 0.9608 0.937]);
      | set(gca, 'gridcolor',[0 0.6902 0.3137]);
      mask Callback Tins2:
      | % Plotting IDMT Curve
      | clf('reset')
      | TMS = str2num(get_param(gcb,'TMS2'));
      | Vp = str2num(get_param(gcb,'Vp'));
      | PS=str2num(get_param(gcb,'PS2'));
      | k = str2num(get_param(gcb,'k2'));
      | alpha = str2num(get_param(gcb,'alpha2'));
      | B = str2num(get_param(gcb,'B2'));
      | Esc = str2num(get_param(gcb,'Esc2'));
      | Tins = str2num(get_param(gcb,'Tins2'));
      | I = [1.1:0.1:Esc];
      | I1=[Esc,Esc:0.1:30];
      | y=((k./((I.^alpha)-1))+B)*TMS;
      | Tin=[((k./((Esc.^alpha)-1))+B)*TMS,ones(1,length(I1)-1)*Tins];
      | loglog(I,y,'r');
      | hold on
      | loglog(I1,Tin,'r');
      | set(gcf, 'Position', [200 150 300 500]);
      | switch(get_param(gcb,'TCpopup2'))
      |     case 'IEC Standard Inverse'
      |         title('IEC Standard Inverse');
      |     case 'IEC Very Inverse'
      |         title('IEC Very Inverse');
      |     case 'IEC Long Time Inverse'
      |         title('IEC Long Time Inverse');
      |     case 'IEC Extremely Inverse'
      |         title('IEC Extremely Inverse');
      |      case 'IEC Ultra Inverse'
      |         title('IEC Ultra Inverse');
      |     case 'IEEE Moderately Inverse'
      |         title('IEEE Moderately Inverse');
      |     case 'IEEE Very Inverse'
      |         title('IEEE Very Inverse');
      |     case 'IEEE Extremely Inverse'
      |         title('IEEE Extremely Inverse');
      | end
      | ymax=10^ceil(log10(max(y)));
      | set(gca, 'XTick',[1:10 20]);
      | set(gca, 'YTick',[0 ymax/1000 ymax/500 ymax/200 ymax/100 ymax/50 ymax/20 ymax/10 ymax/5 ymax/2 ymax]);
      | xlim([0.9 30]);
      | ylim([0.01 ymax]);
      | xlabel(['Corriente multiplicada por Ipick-up(' num2str(PS*Vp) 'A)']);
      | ylabel('Tiempo de Operacion (Seg)');
      | grid on;
      | set(gca, 'color',[0.9608 0.9608 0.937]);
      | set(gca, 'gridcolor',[0 0.6902 0.3137]);
      mask Callback Esc2:
      | % Plotting IDMT Curve
      | clf('reset')
      | TMS = str2num(get_param(gcb,'TMS2'));
      | Vp = str2num(get_param(gcb,'Vp'));
      | PS=str2num(get_param(gcb,'PS2'));
      | k = str2num(get_param(gcb,'k2'));
      | alpha = str2num(get_param(gcb,'alpha2'));
      | B = str2num(get_param(gcb,'B2'));
      | Esc = str2num(get_param(gcb,'Esc2'));
      | Tins = str2num(get_param(gcb,'Tins2'));
      | I = [1.1:0.1:Esc];
      | I1=[Esc,Esc:0.1:30];
      | y=((k./((I.^alpha)-1))+B)*TMS;
      | Tin=[((k./((Esc.^alpha)-1))+B)*TMS,ones(1,length(I1)-1)*Tins];
      | loglog(I,y,'r');
      | hold on
      | loglog(I1,Tin,'r');
      | set(gcf, 'Position', [200 150 300 500]);
      | switch(get_param(gcb,'TCpopup2'))
      |     case 'IEC Standard Inverse'
      |         title('IEC Standard Inverse');
      |     case 'IEC Very Inverse'
      |         title('IEC Very Inverse');
      |     case 'IEC Long Time Inverse'
      |         title('IEC Long Time Inverse');
      |     case 'IEC Extremely Inverse'
      |         title('IEC Extremely Inverse');
      |      case 'IEC Ultra Inverse'
      |         title('IEC Ultra Inverse');
      |     case 'IEEE Moderately Inverse'
      |         title('IEEE Moderately Inverse');
      |     case 'IEEE Very Inverse'
      |         title('IEEE Very Inverse');
      |     case 'IEEE Extremely Inverse'
      |         title('IEEE Extremely Inverse');
      | end
      | ymax=10^ceil(log10(max(y)));
      | set(gca, 'XTick',[1:10 20]);
      | set(gca, 'YTick',[0 ymax/1000 ymax/500 ymax/200 ymax/100 ymax/50 ymax/20 ymax/10 ymax/5 ymax/2 ymax]);
      | xlim([0.9 30]);
      | ylim([0.01 ymax]);
      | xlabel(['Corriente multiplicada por Ipick-up(' num2str(PS*Vp) 'A)']);
      | ylabel('Tiempo de Operacion (Seg)');
      | grid on;
      | set(gca, 'color',[0.9608 0.9608 0.937]);
      | set(gca, 'gridcolor',[0 0.6902 0.3137]);
      mask TypeOptions TCpopup3: IEC Standard Inverse | IEC Very Inverse | IEC Long Time Inverse | IEC Extremely Inverse | IEC Ultra Inverse | IEEE Moderately Inverse | IEEE Very Inverse | IEEE Extremely Inverse
      mask Callback TCpopup3:
      | switch(get_param(gcb,'TCpopup3'))
      |     case 'IEC Standard Inverse'
      |         set_param(gcb,'k3','0.14');
      |         set_param(gcb,'alpha3','0.02');
      |         set_param(gcb,'B3','0');
      |     case 'IEC Very Inverse'
      |         set_param(gcb,'k3','13.5');
      |         set_param(gcb,'alpha3','1');
      |         set_param(gcb,'B3','0');
      |     case 'IEC Long Time Inverse'
      |         set_param(gcb,'k3','120');
      |         set_param(gcb,'alpha3','1');
      |         set_param(gcb,'B3','0');
      |     case 'IEC Extremely Inverse'
      |         set_param(gcb,'k3','80');
      |         set_param(gcb,'alpha3','2');
      |         set_param(gcb,'B3','0');
      |     case 'IEC Ultra Inverse'
      |         set_param(gcb,'k3','315.2');
      |         set_param(gcb,'alpha3','2.5');
      |         set_param(gcb,'B3','0');
      |     case 'IEEE Moderately Inverse'
      |         set_param(gcb,'k3','0.0515');
      |         set_param(gcb,'alpha3','0.02');
      |         set_param(gcb,'B3','0.114');
      |     case 'IEEE Very Inverse'
      |         set_param(gcb,'k3','19.61');
      |         set_param(gcb,'alpha3','2');
      |         set_param(gcb,'B3','0.491');
      |     case 'IEEE Extremely Inverse'
      |         set_param(gcb,'k3','28.2');
      |         set_param(gcb,'alpha3','2');
      |         set_param(gcb,'B3','0.1217');
      | end
      | % Plotting IDMT Curve
      | clf('reset')
      | TMS = str2num(get_param(gcb,'TMS3'));
      | Vp = str2num(get_param(gcb,'Vp'));
      | PS=str2num(get_param(gcb,'PS3'));
      | k = str2num(get_param(gcb,'k3'));
      | alpha = str2num(get_param(gcb,'alpha3'));
      | B = str2num(get_param(gcb,'B3'));
      | Esc = str2num(get_param(gcb,'Esc3'));
      | Tins = str2num(get_param(gcb,'Tins3'));
      | I = [1.1:0.1:Esc];
      | I1=[Esc,Esc:0.1:30];
      | y=((k./((I.^alpha)-1))+B)*TMS;
      | Tin=[((k./((Esc.^alpha)-1))+B)*TMS,ones(1,length(I1)-1)*Tins];
      | loglog(I,y,'m');
      | hold on
      | loglog(I1,Tin,'m');
      | set(gcf, 'Position', [200 150 300 500]);
      | switch(get_param(gcb,'TCpopup3'))
      |     case 'IEC Standard Inverse'
      |         title('IEC Standard Inverse');
      |     case 'IEC Very Inverse'
      |         title('IEC Very Inverse');
      |     case 'IEC Long Time Inverse'
      |         title('IEC Long Time Inverse');
      |     case 'IEC Extremely Inverse'
      |         title('IEC Extremely Inverse');
      |      case 'IEC Ultra Inverse'
      |         title('IEC Ultra Inverse');
      |     case 'IEEE Moderately Inverse'
      |         title('IEEE Moderately Inverse');
      |     case 'IEEE Very Inverse'
      |         title('IEEE Very Inverse');
      |     case 'IEEE Extremely Inverse'
      |         title('IEEE Extremely Inverse');
      | end
      | ymax=10^ceil(log10(max(y)));
      | set(gca, 'XTick',[1:10 20]);
      | set(gca, 'YTick',[0 ymax/1000 ymax/500 ymax/200 ymax/100 ymax/50 ymax/20 ymax/10 ymax/5 ymax/2 ymax]);
      | xlim([0.9 30]);
      | ylim([0.01 ymax]);
      | xlabel(['Corriente multiplicada por Ipick-up(' num2str(PS*Vp) 'A)']);
      | ylabel('Tiempo de Operacion (Seg)');
      | grid on;
      | set(gca, 'color',[0.9608 0.9608 0.937]);
      | set(gca, 'gridcolor',[0 0.6902 0.3137]);
      mask Callback PS3:
      | % Plotting IDMT Curve
      | clf('reset')
      | TMS = str2num(get_param(gcb,'TMS3'));
      | Vp = str2num(get_param(gcb,'Vp'));
      | PS=str2num(get_param(gcb,'PS3'));
      | k = str2num(get_param(gcb,'k3'));
      | alpha = str2num(get_param(gcb,'alpha3'));
      | B = str2num(get_param(gcb,'B3'));
      | Esc = str2num(get_param(gcb,'Esc3'));
      | Tins = str2num(get_param(gcb,'Tins3'));
      | I = [1.1:0.1:Esc];
      | I1=[Esc,Esc:0.1:30];
      | y=((k./((I.^alpha)-1))+B)*TMS;
      | Tin=[((k./((Esc.^alpha)-1))+B)*TMS,ones(1,length(I1)-1)*Tins];
      | loglog(I,y,'m');
      | hold on
      | loglog(I1,Tin,'m');
      | set(gcf, 'Position', [200 150 300 500]);
      | switch(get_param(gcb,'TCpopup3'))
      |     case 'IEC Standard Inverse'
      |         title('IEC Standard Inverse');
      |     case 'IEC Very Inverse'
      |         title('IEC Very Inverse');
      |     case 'IEC Long Time Inverse'
      |         title('IEC Long Time Inverse');
      |     case 'IEC Extremely Inverse'
      |         title('IEC Extremely Inverse');
      |      case 'IEC Ultra Inverse'
      |         title('IEC Ultra Inverse');
      |     case 'IEEE Moderately Inverse'
      |         title('IEEE Moderately Inverse');
      |     case 'IEEE Very Inverse'
      |         title('IEEE Very Inverse');
      |     case 'IEEE Extremely Inverse'
      |         title('IEEE Extremely Inverse');
      | end
      | ymax=10^ceil(log10(max(y)));
      | set(gca, 'XTick',[1:10 20]);
      | set(gca, 'YTick',[0 ymax/1000 ymax/500 ymax/200 ymax/100 ymax/50 ymax/20 ymax/10 ymax/5 ymax/2 ymax]);
      | xlim([0.9 30]);
      | ylim([0.01 ymax]);
      | xlabel(['Corriente multiplicada por Ipick-up(' num2str(PS*Vp) 'A)']);
      | ylabel('Tiempo de Operacion (Seg)');
      | grid on;
      | set(gca, 'color',[0.9608 0.9608 0.937]);
      | set(gca, 'gridcolor',[0 0.6902 0.3137]);
      mask Callback TMS3:
      | % Plotting IDMT Curve
      | clf('reset')
      | TMS = str2num(get_param(gcb,'TMS3'));
      | Vp = str2num(get_param(gcb,'Vp'));
      | PS=str2num(get_param(gcb,'PS3'));
      | k = str2num(get_param(gcb,'k3'));
      | alpha = str2num(get_param(gcb,'alpha3'));
      | B = str2num(get_param(gcb,'B3'));
      | Esc = str2num(get_param(gcb,'Esc3'));
      | Tins = str2num(get_param(gcb,'Tins3'));
      | I = [1.1:0.1:Esc];
      | I1=[Esc,Esc:0.1:30];
      | y=((k./((I.^alpha)-1))+B)*TMS;
      | Tin=[((k./((Esc.^alpha)-1))+B)*TMS,ones(1,length(I1)-1)*Tins];
      | loglog(I,y,'m');
      | hold on
      | loglog(I1,Tin,'m');
      | set(gcf, 'Position', [200 150 300 500]);
      | switch(get_param(gcb,'TCpopup3'))
      |     case 'IEC Standard Inverse'
      |         title('IEC Standard Inverse');
      |     case 'IEC Very Inverse'
      |         title('IEC Very Inverse');
      |     case 'IEC Long Time Inverse'
      |         title('IEC Long Time Inverse');
      |     case 'IEC Extremely Inverse'
      |         title('IEC Extremely Inverse');
      |      case 'IEC Ultra Inverse'
      |         title('IEC Ultra Inverse');
      |     case 'IEEE Moderately Inverse'
      |         title('IEEE Moderately Inverse');
      |     case 'IEEE Very Inverse'
      |         title('IEEE Very Inverse');
      |     case 'IEEE Extremely Inverse'
      |         title('IEEE Extremely Inverse');
      | end
      | ymax=10^ceil(log10(max(y)));
      | set(gca, 'XTick',[1:10 20]);
      | set(gca, 'YTick',[0 ymax/1000 ymax/500 ymax/200 ymax/100 ymax/50 ymax/20 ymax/10 ymax/5 ymax/2 ymax]);
      | xlim([0.9 30]);
      | ylim([0.01 ymax]);
      | xlabel(['Corriente multiplicada por Ipick-up(' num2str(PS*Vp) 'A)']);
      | ylabel('Tiempo de Operacion (Seg)');
      | grid on;
      | set(gca, 'color',[0.9608 0.9608 0.937]);
      | set(gca, 'gridcolor',[0 0.6902 0.3137]);
      mask Callback Tins3:
      | % Plotting IDMT Curve
      | clf('reset')
      | TMS = str2num(get_param(gcb,'TMS3'));
      | Vp = str2num(get_param(gcb,'Vp'));
      | PS=str2num(get_param(gcb,'PS3'));
      | k = str2num(get_param(gcb,'k3'));
      | alpha = str2num(get_param(gcb,'alpha3'));
      | B = str2num(get_param(gcb,'B3'));
      | Esc = str2num(get_param(gcb,'Esc3'));
      | Tins = str2num(get_param(gcb,'Tins3'));
      | I = [1.1:0.1:Esc];
      | I1=[Esc,Esc:0.1:30];
      | y=((k./((I.^alpha)-1))+B)*TMS;
      | Tin=[((k./((Esc.^alpha)-1))+B)*TMS,ones(1,length(I1)-1)*Tins];
      | loglog(I,y,'m');
      | hold on
      | loglog(I1,Tin,'m');
      | set(gcf, 'Position', [200 150 300 500]);
      | switch(get_param(gcb,'TCpopup3'))
      |     case 'IEC Standard Inverse'
      |         title('IEC Standard Inverse');
      |     case 'IEC Very Inverse'
      |         title('IEC Very Inverse');
      |     case 'IEC Long Time Inverse'
      |         title('IEC Long Time Inverse');
      |     case 'IEC Extremely Inverse'
      |         title('IEC Extremely Inverse');
      |      case 'IEC Ultra Inverse'
      |         title('IEC Ultra Inverse');
      |     case 'IEEE Moderately Inverse'
      |         title('IEEE Moderately Inverse');
      |     case 'IEEE Very Inverse'
      |         title('IEEE Very Inverse');
      |     case 'IEEE Extremely Inverse'
      |         title('IEEE Extremely Inverse');
      | end
      | ymax=10^ceil(log10(max(y)));
      | set(gca, 'XTick',[1:10 20]);
      | set(gca, 'YTick',[0 ymax/1000 ymax/500 ymax/200 ymax/100 ymax/50 ymax/20 ymax/10 ymax/5 ymax/2 ymax]);
      | xlim([0.9 30]);
      | ylim([0.01 ymax]);
      | xlabel(['Corriente multiplicada por Ipick-up(' num2str(PS*Vp) 'A)']);
      | ylabel('Tiempo de Operacion (Seg)');
      | grid on;
      | set(gca, 'color',[0.9608 0.9608 0.937]);
      | set(gca, 'gridcolor',[0 0.6902 0.3137]);
      mask Callback Esc3:
      | % Plotting IDMT Curve
      | clf('reset')
      | TMS = str2num(get_param(gcb,'TMS3'));
      | Vp = str2num(get_param(gcb,'Vp'));
      | PS=str2num(get_param(gcb,'PS3'));
      | k = str2num(get_param(gcb,'k3'));
      | alpha = str2num(get_param(gcb,'alpha3'));
      | B = str2num(get_param(gcb,'B3'));
      | Esc = str2num(get_param(gcb,'Esc3'));
      | Tins = str2num(get_param(gcb,'Tins3'));
      | I = [1.1:0.1:Esc];
      | I1=[Esc,Esc:0.1:30];
      | y=((k./((I.^alpha)-1))+B)*TMS;
      | Tin=[((k./((Esc.^alpha)-1))+B)*TMS,ones(1,length(I1)-1)*Tins];
      | loglog(I,y,'m');
      | hold on
      | loglog(I1,Tin,'m');
      | set(gcf, 'Position', [200 150 300 500]);
      | switch(get_param(gcb,'TCpopup3'))
      |     case 'IEC Standard Inverse'
      |         title('IEC Standard Inverse');
      |     case 'IEC Very Inverse'
      |         title('IEC Very Inverse');
      |     case 'IEC Long Time Inverse'
      |         title('IEC Long Time Inverse');
      |     case 'IEC Extremely Inverse'
      |         title('IEC Extremely Inverse');
      |      case 'IEC Ultra Inverse'
      |         title('IEC Ultra Inverse');
      |     case 'IEEE Moderately Inverse'
      |         title('IEEE Moderately Inverse');
      |     case 'IEEE Very Inverse'
      |         title('IEEE Very Inverse');
      |     case 'IEEE Extremely Inverse'
      |         title('IEEE Extremely Inverse');
      | end
      | ymax=10^ceil(log10(max(y)));
      | set(gca, 'XTick',[1:10 20]);
      | set(gca, 'YTick',[0 ymax/1000 ymax/500 ymax/200 ymax/100 ymax/50 ymax/20 ymax/10 ymax/5 ymax/2 ymax]);
      | xlim([0.9 30]);
      | ylim([0.01 ymax]);
      | xlabel(['Corriente multiplicada por Ipick-up(' num2str(PS*Vp) 'A)']);
      | ylabel('Tiempo de Operacion (Seg)');
      | grid on;
      | set(gca, 'color',[0.9608 0.9608 0.937]);
      | set(gca, 'gridcolor',[0 0.6902 0.3137]);
      mask DialogControl Container6 Prompt: Protecciones
      mask DialogControl Container8 Prompt: Topologia 1
      mask DialogControl Container9 Prompt: Proteccion 51
      mask DialogControl Container10 Prompt: Proteccion 50
      mask DialogControl Container8_copy Prompt: Topologia 2
      mask DialogControl Container9_copy Prompt: Proteccion 51
      mask DialogControl Container10_copy Prompt: Proteccion 50
      mask DialogControl Container8_copy_copy Prompt: Topologia 3
      mask DialogControl Container9_copy_copy Prompt: Proteccion 51
      mask DialogControl Container10_copy_copy Prompt: Proteccion 50
      mask DialogControl Container17 Prompt: Caracteristicas Trafo Corriente
      mask Display:
      | port_label('input',1,'D');
      | port_label('input',2,'I');
      | port_label('output',1,'S');
      | text(0.62, 0.5,'50', 'horizontalAlignment', 'center');
      | text(0.62, 0.3,'51', 'horizontalAlignment', 'center');
      | plot([0.08:0.01:0.32]+0.4,[0:0.01:0.24]*0+0.40);
      | plot(0.25*sin([0:pi/20:2*pi])+0.6,0.25*cos([0:pi/20:2*pi])+0.4);
      | %Linea Salida
      | plot([0.85:0.01:1],[0:0.01:0.15]*0+0.4);
      | %Linea Corriente
      | plot([0.2:0.01:0.35],[0:0.01:0.15]*0+0.4);
      | plot([0.1:0.01:0.2],[0:0.01:0.1]*0+0.15);
      | plot([0.1:0.01:0.35]*0+0.2,[0:0.01:0.25]+0.15);
      | %Linea tension
      | plot([0.15:0.01:0.6],[0:0.01:0.45]*0+0.7);
      | plot([0:0.01:0.05]*0+0.6,[0:0.01:0.05]+0.65);
  RB4 : Subsystem  mask(Proteccion de Sobrecorriente multitopologia){menu=3, TCpopup1=IEC Standard Inverse, k1=0.14, alpha1=0.02, B1=0, PS1=0.1, TMS1=0.712, Tins1=0.12, Esc1=12, TCpopup2=IEC Standard Inverse, k2=0.14, alpha2=0.02, B2=0, PS2=1, TMS2=0.150, Tins2=0.2, Esc2=6, TCpopup3=IEC Standard Inverse, k3=0.14, alpha3=0.02, B3=0, PS3=0.6267, TMS3=0.15, Tins3=0.15, Esc3=5, Vp=1200, Vs=5, F=60}
      mask prompts: menu "Numero de Topologias"; TCpopup1 "Caracteristica de Disparo"; k1 "k"; alpha1 "alpha"; B1 "B"; PS1 "Seteo disparo(PS)/Seteo inferior(I>)"; TMS1 "Multiplicador de Tiempo"; Tins1 "Tins"; Esc1 "Escala"; TCpopup2 "Caracteristica de Disparo"; k2 "k"; alpha2 "alpha"; B2 "B"; PS2 "Seteo disparo(PS)/Seteo inferior(I>)"; TMS2 "Multiplicador de tiempo"; Tins2 "Tins"; Esc2 "Escala"; TCpopup3 "Caracteristica de Disparo"; k3 "k"; alpha3 "alpha"; B3 "B"; PS3 "Seteo disparo(PS)/Seteo inferior(I>)"; TMS3 "Multiplicador de Tiempo"; Tins3 "Tins"; Esc3 "Escala"; Vp "Primario CT"; Vs "Secundario CT"; F "Frecuencia"
      mask help: Proteccion de Sobrecorriente con tres topologias internas controladas por una señal de control externa.
      mask init:
      | warning('off','Simulink:Masking:Invalid_Visible_Flag')
      mask TypeOptions menu: 1 | 2 | 3
      mask Callback menu:
      | h = getSimulinkBlockHandle(gcb);
      | menu1 = get_param(h,'menu');
      | if strcmp(menu1,num2str(1))
      |     set_param(h,'MaskVisibilities',{'on',...
      |         'on','on','on','on','on','on','on','on',...%proteccion 1 activa
      |         'off','off','off','off','off','off','off','off',...%proteccion 2 desactivada
      |         'off','off','off','off','off','off','off','off',...%proteccion 3 desactivada
      |         'on','on','on'});%Otros parametros activados
      |     Int=1;
      | elseif strcmp(menu1,num2str(2))
      |  set_param(h,'MaskVisibilities',{'on',...
      |         'on','on','on','on','on','on','on','on',...%proteccion 1 activa
      |         'on','on','on','on','on','on','on','on',...%proteccion 2 activa
      |         'off','off','off','off','off','off','off','off',...%proteccion 3 desactivada
      |         'on','on','on'});%Otros parametros activados
      |     Int=2;
      | else
      | set_param(h,'MaskVisibilities',{'on',...
      |         'on','on','on','on','on','on','on','on',...%proteccion 1 activa
      |         'on','on','on','on','on','on','on','on',...%proteccion 2 activa
      |         'on','on','on','on','on','on','on','on',...%proteccion 3 desactivada
      |         'on','on','on'});%Otros parametros activados
      |     Int=3;
      | end
      mask TypeOptions TCpopup1: IEC Standard Inverse | IEC Very Inverse | IEC Long Time Inverse | IEC Extremely Inverse | IEC Ultra Inverse | IEEE Moderately Inverse | IEEE Very Inverse | IEEE Extremely Inverse
      mask Callback TCpopup1:
      | switch(get_param(gcb,'TCpopup1'))
      |     case 'IEC Standard Inverse'
      |         set_param(gcb,'k1','0.14');
      |         set_param(gcb,'alpha1','0.02');
      |         set_param(gcb,'B1','0');
      |     case 'IEC Very Inverse'
      |         set_param(gcb,'k1','13.5');
      |         set_param(gcb,'alpha1','1');
      |         set_param(gcb,'B1','0');
      |     case 'IEC Long Time Inverse'
      |         set_param(gcb,'k1','120');
      |         set_param(gcb,'alpha1','1');
      |         set_param(gcb,'B1','0');
      |     case 'IEC Extremely Inverse'
      |         set_param(gcb,'k1','80');
      |         set_param(gcb,'alpha1','2');
      |         set_param(gcb,'B1','0');
      |     case 'IEC Ultra Inverse'
      |         set_param(gcb,'k1','315.2');
      |         set_param(gcb,'alpha1','2.5');
      |         set_param(gcb,'B1','0');
      |     case 'IEEE Moderately Inverse'
      |         set_param(gcb,'k1','0.0515');
      |         set_param(gcb,'alpha1','0.02');
      |         set_param(gcb,'B1','0.114');
      |     case 'IEEE Very Inverse'
      |         set_param(gcb,'k1','19.61');
      |         set_param(gcb,'alpha1','2');
      |         set_param(gcb,'B1','0.491');
      |     case 'IEEE Extremely Inverse'
      |         set_param(gcb,'k1','28.2');
      |         set_param(gcb,'alpha1','2');
      |         set_param(gcb,'B1','0.1217');
      | end
      | % Plotting IDMT Curve
      | clf('reset')
      | TMS = str2num(get_param(gcb,'TMS1'));
      | Vp = str2num(get_param(gcb,'Vp'));
      | PS=str2num(get_param(gcb,'PS1'));
      | k = str2num(get_param(gcb,'k1'));
      | alpha = str2num(get_param(gcb,'alpha1'));
      | B = str2num(get_param(gcb,'B1'));
      | Esc = str2num(get_param(gcb,'Esc1'));
      | Tins = str2num(get_param(gcb,'Tins1'));
      | I = [1.1:0.1:Esc];
      | I1=[Esc,Esc:0.1:30];
      | y=((k./((I.^alpha)-1))+B)*TMS;
      | Tin=[((k./((Esc.^alpha)-1))+B)*TMS,ones(1,length(I1)-1)*Tins];
      | loglog(I,y,'b');
      | hold on
      | loglog(I1,Tin,'b');
      | set(gcf, 'Position', [200 150 300 500]);
      | switch(get_param(gcb,'TCpopup1'))
      |     case 'IEC Standard Inverse'
      |         title('IEC Standard Inverse');
      |     case 'IEC Very Inverse'
      |         title('IEC Very Inverse');
      |     case 'IEC Long Time Inverse'
      |         title('IEC Long Time Inverse');
      |     case 'IEC Extremely Inverse'
      |         title('IEC Extremely Inverse');
      |      case 'IEC Ultra Inverse'
      |         title('IEC Ultra Inverse');
      |     case 'IEEE Moderately Inverse'
      |         title('IEEE Moderately Inverse');
      |     case 'IEEE Very Inverse'
      |         title('IEEE Very Inverse');
      |     case 'IEEE Extremely Inverse'
      |         title('IEEE Extremely Inverse');
      | end
      | ymax=10^ceil(log10(max(y)));
      | set(gca, 'XTick',[1:10 20]);
      | set(gca, 'YTick',[0 ymax/1000 ymax/500 ymax/200 ymax/100 ymax/50 ymax/20 ymax/10 ymax/5 ymax/2 ymax]);
      | xlim([0.9 30]);
      | ylim([0.01 ymax]);
      | xlabel(['Corriente multiplicada por Ipick-up(' num2str(PS*Vp) 'A)']);
      | ylabel('Tiempo de Operacion (Seg)');
      | grid on;
      | set(gca, 'color',[0.9608 0.9608 0.937]);
      | set(gca, 'gridcolor',[0 0.6902 0.3137]);
      mask Callback PS1:
      | % Plotting IDMT Curve
      | clf('reset')
      | TMS = str2num(get_param(gcb,'TMS1'));
      | Vp = str2num(get_param(gcb,'Vp'));
      | PS=str2num(get_param(gcb,'PS1'));
      | k = str2num(get_param(gcb,'k1'));
      | alpha = str2num(get_param(gcb,'alpha1'));
      | B = str2num(get_param(gcb,'B1'));
      | Esc = str2num(get_param(gcb,'Esc1'));
      | Tins = str2num(get_param(gcb,'Tins1'));
      | I = [1.1:0.1:Esc];
      | I1=[Esc,Esc:0.1:30];
      | y=((k./((I.^alpha)-1))+B)*TMS;
      | Tin=[((k./((Esc.^alpha)-1))+B)*TMS,ones(1,length(I1)-1)*Tins];
      | loglog(I,y,'b');
      | hold on
      | loglog(I1,Tin,'b');
      | set(gcf, 'Position', [200 150 300 500]);
      | switch(get_param(gcb,'TCpopup1'))
      |     case 'IEC Standard Inverse'
      |         title('IEC Standard Inverse');
      |     case 'IEC Very Inverse'
      |         title('IEC Very Inverse');
      |     case 'IEC Long Time Inverse'
      |         title('IEC Long Time Inverse');
      |     case 'IEC Extremely Inverse'
      |         title('IEC Extremely Inverse');
      |      case 'IEC Ultra Inverse'
      |         title('IEC Ultra Inverse');
      |     case 'IEEE Moderately Inverse'
      |         title('IEEE Moderately Inverse');
      |     case 'IEEE Very Inverse'
      |         title('IEEE Very Inverse');
      |     case 'IEEE Extremely Inverse'
      |         title('IEEE Extremely Inverse');
      | end
      | ymax=10^ceil(log10(max(y)));
      | set(gca, 'XTick',[1:10 20]);
      | set(gca, 'YTick',[0 ymax/1000 ymax/500 ymax/200 ymax/100 ymax/50 ymax/20 ymax/10 ymax/5 ymax/2 ymax]);
      | xlim([0.9 30]);
      | ylim([0.01 ymax]);
      | xlabel(['Corriente multiplicada por Ipick-up(' num2str(PS*Vp) 'A)']);
      | ylabel('Tiempo de Operacion (Seg)');
      | grid on;
      | set(gca, 'color',[0.9608 0.9608 0.937]);
      | set(gca, 'gridcolor',[0 0.6902 0.3137]);
      mask Callback TMS1:
      | % Plotting IDMT Curve
      | clf('reset')
      | TMS = str2num(get_param(gcb,'TMS1'));
      | Vp = str2num(get_param(gcb,'Vp'));
      | PS=str2num(get_param(gcb,'PS1'));
      | k = str2num(get_param(gcb,'k1'));
      | alpha = str2num(get_param(gcb,'alpha1'));
      | B = str2num(get_param(gcb,'B1'));
      | Esc = str2num(get_param(gcb,'Esc1'));
      | Tins = str2num(get_param(gcb,'Tins1'));
      | I = [1.1:0.1:Esc];
      | I1=[Esc,Esc:0.1:30];
      | y=((k./((I.^alpha)-1))+B)*TMS;
      | Tin=[((k./((Esc.^alpha)-1))+B)*TMS,ones(1,length(I1)-1)*Tins];
      | loglog(I,y,'b');
      | hold on
      | loglog(I1,Tin,'b');
      | set(gcf, 'Position', [200 150 300 500]);
      | switch(get_param(gcb,'TCpopup1'))
      |     case 'IEC Standard Inverse'
      |         title('IEC Standard Inverse');
      |     case 'IEC Very Inverse'
      |         title('IEC Very Inverse');
      |     case 'IEC Long Time Inverse'
      |         title('IEC Long Time Inverse');
      |     case 'IEC Extremely Inverse'
      |         title('IEC Extremely Inverse');
      |      case 'IEC Ultra Inverse'
      |         title('IEC Ultra Inverse');
      |     case 'IEEE Moderately Inverse'
      |         title('IEEE Moderately Inverse');
      |     case 'IEEE Very Inverse'
      |         title('IEEE Very Inverse');
      |     case 'IEEE Extremely Inverse'
      |         title('IEEE Extremely Inverse');
      | end
      | ymax=10^ceil(log10(max(y)));
      | set(gca, 'XTick',[1:10 20]);
      | set(gca, 'YTick',[0 ymax/1000 ymax/500 ymax/200 ymax/100 ymax/50 ymax/20 ymax/10 ymax/5 ymax/2 ymax]);
      | xlim([0.9 30]);
      | ylim([0.01 ymax]);
      | xlabel(['Corriente multiplicada por Ipick-up(' num2str(PS*Vp) 'A)']);
      | ylabel('Tiempo de Operacion (Seg)');
      | grid on;
      | set(gca, 'color',[0.9608 0.9608 0.937]);
      | set(gca, 'gridcolor',[0 0.6902 0.3137]);
      mask Callback Tins1:
      | % Plotting IDMT Curve
      | clf('reset')
      | TMS = str2num(get_param(gcb,'TMS1'));
      | Vp = str2num(get_param(gcb,'Vp'));
      | PS=str2num(get_param(gcb,'PS1'));
      | k = str2num(get_param(gcb,'k1'));
      | alpha = str2num(get_param(gcb,'alpha1'));
      | B = str2num(get_param(gcb,'B1'));
      | Esc = str2num(get_param(gcb,'Esc1'));
      | Tins = str2num(get_param(gcb,'Tins1'));
      | I = [1.1:0.1:Esc];
      | I1=[Esc,Esc:0.1:30];
      | y=((k./((I.^alpha)-1))+B)*TMS;
      | Tin=[((k./((Esc.^alpha)-1))+B)*TMS,ones(1,length(I1)-1)*Tins];
      | loglog(I,y,'b');
      | hold on
      | loglog(I1,Tin,'b');
      | set(gcf, 'Position', [200 150 300 500]);
      | switch(get_param(gcb,'TCpopup1'))
      |     case 'IEC Standard Inverse'
      |         title('IEC Standard Inverse');
      |     case 'IEC Very Inverse'
      |         title('IEC Very Inverse');
      |     case 'IEC Long Time Inverse'
      |         title('IEC Long Time Inverse');
      |     case 'IEC Extremely Inverse'
      |         title('IEC Extremely Inverse');
      |      case 'IEC Ultra Inverse'
      |         title('IEC Ultra Inverse');
      |     case 'IEEE Moderately Inverse'
      |         title('IEEE Moderately Inverse');
      |     case 'IEEE Very Inverse'
      |         title('IEEE Very Inverse');
      |     case 'IEEE Extremely Inverse'
      |         title('IEEE Extremely Inverse');
      | end
      | ymax=10^ceil(log10(max(y)));
      | set(gca, 'XTick',[1:10 20]);
      | set(gca, 'YTick',[0 ymax/1000 ymax/500 ymax/200 ymax/100 ymax/50 ymax/20 ymax/10 ymax/5 ymax/2 ymax]);
      | xlim([0.9 30]);
      | ylim([0.01 ymax]);
      | xlabel(['Corriente multiplicada por Ipick-up(' num2str(PS*Vp) 'A)']);
      | ylabel('Tiempo de Operacion (Seg)');
      | grid on;
      | set(gca, 'color',[0.9608 0.9608 0.937]);
      | set(gca, 'gridcolor',[0 0.6902 0.3137]);
      mask Callback Esc1:
      | % Plotting IDMT Curve
      | clf('reset')
      | TMS = str2num(get_param(gcb,'TMS1'));
      | Vp = str2num(get_param(gcb,'Vp'));
      | PS=str2num(get_param(gcb,'PS1'));
      | k = str2num(get_param(gcb,'k1'));
      | alpha = str2num(get_param(gcb,'alpha1'));
      | B = str2num(get_param(gcb,'B1'));
      | Esc = str2num(get_param(gcb,'Esc1'));
      | Tins = str2num(get_param(gcb,'Tins1'));
      | I = [1.1:0.1:Esc];
      | I1=[Esc,Esc:0.1:30];
      | y=((k./((I.^alpha)-1))+B)*TMS;
      | Tin=[((k./((Esc.^alpha)-1))+B)*TMS,ones(1,length(I1)-1)*Tins];
      | loglog(I,y,'b');
      | hold on
      | loglog(I1,Tin,'b');
      | set(gcf, 'Position', [200 150 300 500]);
      | switch(get_param(gcb,'TCpopup1'))
      |     case 'IEC Standard Inverse'
      |         title('IEC Standard Inverse');
      |     case 'IEC Very Inverse'
      |         title('IEC Very Inverse');
      |     case 'IEC Long Time Inverse'
      |         title('IEC Long Time Inverse');
      |     case 'IEC Extremely Inverse'
      |         title('IEC Extremely Inverse');
      |      case 'IEC Ultra Inverse'
      |         title('IEC Ultra Inverse');
      |     case 'IEEE Moderately Inverse'
      |         title('IEEE Moderately Inverse');
      |     case 'IEEE Very Inverse'
      |         title('IEEE Very Inverse');
      |     case 'IEEE Extremely Inverse'
      |         title('IEEE Extremely Inverse');
      | end
      | ymax=10^ceil(log10(max(y)));
      | set(gca, 'XTick',[1:10 20]);
      | set(gca, 'YTick',[0 ymax/1000 ymax/500 ymax/200 ymax/100 ymax/50 ymax/20 ymax/10 ymax/5 ymax/2 ymax]);
      | xlim([0.9 30]);
      | ylim([0.01 ymax]);
      | xlabel(['Corriente multiplicada por Ipick-up(' num2str(PS*Vp) 'A)']);
      | ylabel('Tiempo de Operacion (Seg)');
      | grid on;
      | set(gca, 'color',[0.9608 0.9608 0.937]);
      | set(gca, 'gridcolor',[0 0.6902 0.3137]);
      mask TypeOptions TCpopup2: IEC Standard Inverse | IEC Very Inverse | IEC Long Time Inverse | IEC Extremely Inverse | IEC Ultra Inverse | IEEE Moderately Inverse | IEEE Very Inverse | IEEE Extremely Inverse
      mask Callback TCpopup2:
      | switch(get_param(gcb,'TCpopup2'))
      |     case 'IEC Standard Inverse'
      |         set_param(gcb,'k2','0.14');
      |         set_param(gcb,'alpha2','0.02');
      |         set_param(gcb,'B2','0');
      |     case 'IEC Very Inverse'
      |         set_param(gcb,'k2','13.5');
      |         set_param(gcb,'alpha2','1');
      |         set_param(gcb,'B2','0');
      |     case 'IEC Long Time Inverse'
      |         set_param(gcb,'k2','120');
      |         set_param(gcb,'alpha2','1');
      |         set_param(gcb,'B2','0');
      |     case 'IEC Extremely Inverse'
      |         set_param(gcb,'k2','80');
      |         set_param(gcb,'alpha2','2');
      |         set_param(gcb,'B2','0');
      |     case 'IEC Ultra Inverse'
      |         set_param(gcb,'k2','315.2');
      |         set_param(gcb,'alpha2','2.5');
      |         set_param(gcb,'B2','0');
      |     case 'IEEE Moderately Inverse'
      |         set_param(gcb,'k2','0.0515');
      |         set_param(gcb,'alpha2','0.02');
      |         set_param(gcb,'B2','0.114');
      |     case 'IEEE Very Inverse'
      |         set_param(gcb,'k2','19.61');
      |         set_param(gcb,'alpha2','2');
      |         set_param(gcb,'B2','0.491');
      |     case 'IEEE Extremely Inverse'
      |         set_param(gcb,'k2','28.2');
      |         set_param(gcb,'alpha2','2');
      |         set_param(gcb,'B2','0.1217');
      | end
      | % Plotting IDMT Curve
      | clf('reset')
      | TMS = str2num(get_param(gcb,'TMS2'));
      | Vp = str2num(get_param(gcb,'Vp'));
      | PS=str2num(get_param(gcb,'PS2'));
      | k = str2num(get_param(gcb,'k2'));
      | alpha = str2num(get_param(gcb,'alpha2'));
      | B = str2num(get_param(gcb,'B2'));
      | Esc = str2num(get_param(gcb,'Esc2'));
      | Tins = str2num(get_param(gcb,'Tins2'));
      | I = [1.1:0.1:Esc];
      | I1=[Esc,Esc:0.1:30];
      | y=((k./((I.^alpha)-1))+B)*TMS;
      | Tin=[((k./((Esc.^alpha)-1))+B)*TMS,ones(1,length(I1)-1)*Tins];
      | loglog(I,y,'r');
      | hold on
      | loglog(I1,Tin,'r');
      | set(gcf, 'Position', [200 150 300 500]);
      | switch(get_param(gcb,'TCpopup2'))
      |     case 'IEC Standard Inverse'
      |         title('IEC Standard Inverse');
      |     case 'IEC Very Inverse'
      |         title('IEC Very Inverse');
      |     case 'IEC Long Time Inverse'
      |         title('IEC Long Time Inverse');
      |     case 'IEC Extremely Inverse'
      |         title('IEC Extremely Inverse');
      |      case 'IEC Ultra Inverse'
      |         title('IEC Ultra Inverse');
      |     case 'IEEE Moderately Inverse'
      |         title('IEEE Moderately Inverse');
      |     case 'IEEE Very Inverse'
      |         title('IEEE Very Inverse');
      |     case 'IEEE Extremely Inverse'
      |         title('IEEE Extremely Inverse');
      | end
      | ymax=10^ceil(log10(max(y)));
      | set(gca, 'XTick',[1:10 20]);
      | set(gca, 'YTick',[0 ymax/1000 ymax/500 ymax/200 ymax/100 ymax/50 ymax/20 ymax/10 ymax/5 ymax/2 ymax]);
      | xlim([0.9 30]);
      | ylim([0.01 ymax]);
      | xlabel(['Corriente multiplicada por Ipick-up(' num2str(PS*Vp) 'A)']);
      | ylabel('Tiempo de Operacion (Seg)');
      | grid on;
      | set(gca, 'color',[0.9608 0.9608 0.937]);
      | set(gca, 'gridcolor',[0 0.6902 0.3137]);
      mask Callback PS2:
      | % Plotting IDMT Curve
      | clf('reset')
      | TMS = str2num(get_param(gcb,'TMS2'));
      | Vp = str2num(get_param(gcb,'Vp'));
      | PS=str2num(get_param(gcb,'PS2'));
      | k = str2num(get_param(gcb,'k2'));
      | alpha = str2num(get_param(gcb,'alpha2'));
      | B = str2num(get_param(gcb,'B2'));
      | Esc = str2num(get_param(gcb,'Esc2'));
      | Tins = str2num(get_param(gcb,'Tins2'));
      | I = [1.1:0.1:Esc];
      | I1=[Esc,Esc:0.1:30];
      | y=((k./((I.^alpha)-1))+B)*TMS;
      | Tin=[((k./((Esc.^alpha)-1))+B)*TMS,ones(1,length(I1)-1)*Tins];
      | loglog(I,y,'r');
      | hold on
      | loglog(I1,Tin,'r');
      | set(gcf, 'Position', [200 150 300 500]);
      | switch(get_param(gcb,'TCpopup2'))
      |     case 'IEC Standard Inverse'
      |         title('IEC Standard Inverse');
      |     case 'IEC Very Inverse'
      |         title('IEC Very Inverse');
      |     case 'IEC Long Time Inverse'
      |         title('IEC Long Time Inverse');
      |     case 'IEC Extremely Inverse'
      |         title('IEC Extremely Inverse');
      |      case 'IEC Ultra Inverse'
      |         title('IEC Ultra Inverse');
      |     case 'IEEE Moderately Inverse'
      |         title('IEEE Moderately Inverse');
      |     case 'IEEE Very Inverse'
      |         title('IEEE Very Inverse');
      |     case 'IEEE Extremely Inverse'
      |         title('IEEE Extremely Inverse');
      | end
      | ymax=10^ceil(log10(max(y)));
      | set(gca, 'XTick',[1:10 20]);
      | set(gca, 'YTick',[0 ymax/1000 ymax/500 ymax/200 ymax/100 ymax/50 ymax/20 ymax/10 ymax/5 ymax/2 ymax]);
      | xlim([0.9 30]);
      | ylim([0.01 ymax]);
      | xlabel(['Corriente multiplicada por Ipick-up(' num2str(PS*Vp) 'A)']);
      | ylabel('Tiempo de Operacion (Seg)');
      | grid on;
      | set(gca, 'color',[0.9608 0.9608 0.937]);
      | set(gca, 'gridcolor',[0 0.6902 0.3137]);
      mask Callback TMS2:
      | % Plotting IDMT Curve
      | clf('reset')
      | TMS = str2num(get_param(gcb,'TMS2'));
      | Vp = str2num(get_param(gcb,'Vp'));
      | PS=str2num(get_param(gcb,'PS2'));
      | k = str2num(get_param(gcb,'k2'));
      | alpha = str2num(get_param(gcb,'alpha2'));
      | B = str2num(get_param(gcb,'B2'));
      | Esc = str2num(get_param(gcb,'Esc2'));
      | Tins = str2num(get_param(gcb,'Tins2'));
      | I = [1.1:0.1:Esc];
      | I1=[Esc,Esc:0.1:30];
      | y=((k./((I.^alpha)-1))+B)*TMS;
      | Tin=[((k./((Esc.^alpha)-1))+B)*TMS,ones(1,length(I1)-1)*Tins];
      | loglog(I,y,'r');
      | hold on
      | loglog(I1,Tin,'r');
      | set(gcf, 'Position', [200 150 300 500]);
      | switch(get_param(gcb,'TCpopup2'))
      |     case 'IEC Standard Inverse'
      |         title('IEC Standard Inverse');
      |     case 'IEC Very Inverse'
      |         title('IEC Very Inverse');
      |     case 'IEC Long Time Inverse'
      |         title('IEC Long Time Inverse');
      |     case 'IEC Extremely Inverse'
      |         title('IEC Extremely Inverse');
      |      case 'IEC Ultra Inverse'
      |         title('IEC Ultra Inverse');
      |     case 'IEEE Moderately Inverse'
      |         title('IEEE Moderately Inverse');
      |     case 'IEEE Very Inverse'
      |         title('IEEE Very Inverse');
      |     case 'IEEE Extremely Inverse'
      |         title('IEEE Extremely Inverse');
      | end
      | ymax=10^ceil(log10(max(y)));
      | set(gca, 'XTick',[1:10 20]);
      | set(gca, 'YTick',[0 ymax/1000 ymax/500 ymax/200 ymax/100 ymax/50 ymax/20 ymax/10 ymax/5 ymax/2 ymax]);
      | xlim([0.9 30]);
      | ylim([0.01 ymax]);
      | xlabel(['Corriente multiplicada por Ipick-up(' num2str(PS*Vp) 'A)']);
      | ylabel('Tiempo de Operacion (Seg)');
      | grid on;
      | set(gca, 'color',[0.9608 0.9608 0.937]);
      | set(gca, 'gridcolor',[0 0.6902 0.3137]);
      mask Callback Tins2:
      | % Plotting IDMT Curve
      | clf('reset')
      | TMS = str2num(get_param(gcb,'TMS2'));
      | Vp = str2num(get_param(gcb,'Vp'));
      | PS=str2num(get_param(gcb,'PS2'));
      | k = str2num(get_param(gcb,'k2'));
      | alpha = str2num(get_param(gcb,'alpha2'));
      | B = str2num(get_param(gcb,'B2'));
      | Esc = str2num(get_param(gcb,'Esc2'));
      | Tins = str2num(get_param(gcb,'Tins2'));
      | I = [1.1:0.1:Esc];
      | I1=[Esc,Esc:0.1:30];
      | y=((k./((I.^alpha)-1))+B)*TMS;
      | Tin=[((k./((Esc.^alpha)-1))+B)*TMS,ones(1,length(I1)-1)*Tins];
      | loglog(I,y,'r');
      | hold on
      | loglog(I1,Tin,'r');
      | set(gcf, 'Position', [200 150 300 500]);
      | switch(get_param(gcb,'TCpopup2'))
      |     case 'IEC Standard Inverse'
      |         title('IEC Standard Inverse');
      |     case 'IEC Very Inverse'
      |         title('IEC Very Inverse');
      |     case 'IEC Long Time Inverse'
      |         title('IEC Long Time Inverse');
      |     case 'IEC Extremely Inverse'
      |         title('IEC Extremely Inverse');
      |      case 'IEC Ultra Inverse'
      |         title('IEC Ultra Inverse');
      |     case 'IEEE Moderately Inverse'
      |         title('IEEE Moderately Inverse');
      |     case 'IEEE Very Inverse'
      |         title('IEEE Very Inverse');
      |     case 'IEEE Extremely Inverse'
      |         title('IEEE Extremely Inverse');
      | end
      | ymax=10^ceil(log10(max(y)));
      | set(gca, 'XTick',[1:10 20]);
      | set(gca, 'YTick',[0 ymax/1000 ymax/500 ymax/200 ymax/100 ymax/50 ymax/20 ymax/10 ymax/5 ymax/2 ymax]);
      | xlim([0.9 30]);
      | ylim([0.01 ymax]);
      | xlabel(['Corriente multiplicada por Ipick-up(' num2str(PS*Vp) 'A)']);
      | ylabel('Tiempo de Operacion (Seg)');
      | grid on;
      | set(gca, 'color',[0.9608 0.9608 0.937]);
      | set(gca, 'gridcolor',[0 0.6902 0.3137]);
      mask Callback Esc2:
      | % Plotting IDMT Curve
      | clf('reset')
      | TMS = str2num(get_param(gcb,'TMS2'));
      | Vp = str2num(get_param(gcb,'Vp'));
      | PS=str2num(get_param(gcb,'PS2'));
      | k = str2num(get_param(gcb,'k2'));
      | alpha = str2num(get_param(gcb,'alpha2'));
      | B = str2num(get_param(gcb,'B2'));
      | Esc = str2num(get_param(gcb,'Esc2'));
      | Tins = str2num(get_param(gcb,'Tins2'));
      | I = [1.1:0.1:Esc];
      | I1=[Esc,Esc:0.1:30];
      | y=((k./((I.^alpha)-1))+B)*TMS;
      | Tin=[((k./((Esc.^alpha)-1))+B)*TMS,ones(1,length(I1)-1)*Tins];
      | loglog(I,y,'r');
      | hold on
      | loglog(I1,Tin,'r');
      | set(gcf, 'Position', [200 150 300 500]);
      | switch(get_param(gcb,'TCpopup2'))
      |     case 'IEC Standard Inverse'
      |         title('IEC Standard Inverse');
      |     case 'IEC Very Inverse'
      |         title('IEC Very Inverse');
      |     case 'IEC Long Time Inverse'
      |         title('IEC Long Time Inverse');
      |     case 'IEC Extremely Inverse'
      |         title('IEC Extremely Inverse');
      |      case 'IEC Ultra Inverse'
      |         title('IEC Ultra Inverse');
      |     case 'IEEE Moderately Inverse'
      |         title('IEEE Moderately Inverse');
      |     case 'IEEE Very Inverse'
      |         title('IEEE Very Inverse');
      |     case 'IEEE Extremely Inverse'
      |         title('IEEE Extremely Inverse');
      | end
      | ymax=10^ceil(log10(max(y)));
      | set(gca, 'XTick',[1:10 20]);
      | set(gca, 'YTick',[0 ymax/1000 ymax/500 ymax/200 ymax/100 ymax/50 ymax/20 ymax/10 ymax/5 ymax/2 ymax]);
      | xlim([0.9 30]);
      | ylim([0.01 ymax]);
      | xlabel(['Corriente multiplicada por Ipick-up(' num2str(PS*Vp) 'A)']);
      | ylabel('Tiempo de Operacion (Seg)');
      | grid on;
      | set(gca, 'color',[0.9608 0.9608 0.937]);
      | set(gca, 'gridcolor',[0 0.6902 0.3137]);
      mask TypeOptions TCpopup3: IEC Standard Inverse | IEC Very Inverse | IEC Long Time Inverse | IEC Extremely Inverse | IEC Ultra Inverse | IEEE Moderately Inverse | IEEE Very Inverse | IEEE Extremely Inverse
      mask Callback TCpopup3:
      | switch(get_param(gcb,'TCpopup3'))
      |     case 'IEC Standard Inverse'
      |         set_param(gcb,'k3','0.14');
      |         set_param(gcb,'alpha3','0.02');
      |         set_param(gcb,'B3','0');
      |     case 'IEC Very Inverse'
      |         set_param(gcb,'k3','13.5');
      |         set_param(gcb,'alpha3','1');
      |         set_param(gcb,'B3','0');
      |     case 'IEC Long Time Inverse'
      |         set_param(gcb,'k3','120');
      |         set_param(gcb,'alpha3','1');
      |         set_param(gcb,'B3','0');
      |     case 'IEC Extremely Inverse'
      |         set_param(gcb,'k3','80');
      |         set_param(gcb,'alpha3','2');
      |         set_param(gcb,'B3','0');
      |     case 'IEC Ultra Inverse'
      |         set_param(gcb,'k3','315.2');
      |         set_param(gcb,'alpha3','2.5');
      |         set_param(gcb,'B3','0');
      |     case 'IEEE Moderately Inverse'
      |         set_param(gcb,'k3','0.0515');
      |         set_param(gcb,'alpha3','0.02');
      |         set_param(gcb,'B3','0.114');
      |     case 'IEEE Very Inverse'
      |         set_param(gcb,'k3','19.61');
      |         set_param(gcb,'alpha3','2');
      |         set_param(gcb,'B3','0.491');
      |     case 'IEEE Extremely Inverse'
      |         set_param(gcb,'k3','28.2');
      |         set_param(gcb,'alpha3','2');
      |         set_param(gcb,'B3','0.1217');
      | end
      | % Plotting IDMT Curve
      | clf('reset')
      | TMS = str2num(get_param(gcb,'TMS3'));
      | Vp = str2num(get_param(gcb,'Vp'));
      | PS=str2num(get_param(gcb,'PS3'));
      | k = str2num(get_param(gcb,'k3'));
      | alpha = str2num(get_param(gcb,'alpha3'));
      | B = str2num(get_param(gcb,'B3'));
      | Esc = str2num(get_param(gcb,'Esc3'));
      | Tins = str2num(get_param(gcb,'Tins3'));
      | I = [1.1:0.1:Esc];
      | I1=[Esc,Esc:0.1:30];
      | y=((k./((I.^alpha)-1))+B)*TMS;
      | Tin=[((k./((Esc.^alpha)-1))+B)*TMS,ones(1,length(I1)-1)*Tins];
      | loglog(I,y,'m');
      | hold on
      | loglog(I1,Tin,'m');
      | set(gcf, 'Position', [200 150 300 500]);
      | switch(get_param(gcb,'TCpopup3'))
      |     case 'IEC Standard Inverse'
      |         title('IEC Standard Inverse');
      |     case 'IEC Very Inverse'
      |         title('IEC Very Inverse');
      |     case 'IEC Long Time Inverse'
      |         title('IEC Long Time Inverse');
      |     case 'IEC Extremely Inverse'
      |         title('IEC Extremely Inverse');
      |      case 'IEC Ultra Inverse'
      |         title('IEC Ultra Inverse');
      |     case 'IEEE Moderately Inverse'
      |         title('IEEE Moderately Inverse');
      |     case 'IEEE Very Inverse'
      |         title('IEEE Very Inverse');
      |     case 'IEEE Extremely Inverse'
      |         title('IEEE Extremely Inverse');
      | end
      | ymax=10^ceil(log10(max(y)));
      | set(gca, 'XTick',[1:10 20]);
      | set(gca, 'YTick',[0 ymax/1000 ymax/500 ymax/200 ymax/100 ymax/50 ymax/20 ymax/10 ymax/5 ymax/2 ymax]);
      | xlim([0.9 30]);
      | ylim([0.01 ymax]);
      | xlabel(['Corriente multiplicada por Ipick-up(' num2str(PS*Vp) 'A)']);
      | ylabel('Tiempo de Operacion (Seg)');
      | grid on;
      | set(gca, 'color',[0.9608 0.9608 0.937]);
      | set(gca, 'gridcolor',[0 0.6902 0.3137]);
      mask Callback PS3:
      | % Plotting IDMT Curve
      | clf('reset')
      | TMS = str2num(get_param(gcb,'TMS3'));
      | Vp = str2num(get_param(gcb,'Vp'));
      | PS=str2num(get_param(gcb,'PS3'));
      | k = str2num(get_param(gcb,'k3'));
      | alpha = str2num(get_param(gcb,'alpha3'));
      | B = str2num(get_param(gcb,'B3'));
      | Esc = str2num(get_param(gcb,'Esc3'));
      | Tins = str2num(get_param(gcb,'Tins3'));
      | I = [1.1:0.1:Esc];
      | I1=[Esc,Esc:0.1:30];
      | y=((k./((I.^alpha)-1))+B)*TMS;
      | Tin=[((k./((Esc.^alpha)-1))+B)*TMS,ones(1,length(I1)-1)*Tins];
      | loglog(I,y,'m');
      | hold on
      | loglog(I1,Tin,'m');
      | set(gcf, 'Position', [200 150 300 500]);
      | switch(get_param(gcb,'TCpopup3'))
      |     case 'IEC Standard Inverse'
      |         title('IEC Standard Inverse');
      |     case 'IEC Very Inverse'
      |         title('IEC Very Inverse');
      |     case 'IEC Long Time Inverse'
      |         title('IEC Long Time Inverse');
      |     case 'IEC Extremely Inverse'
      |         title('IEC Extremely Inverse');
      |      case 'IEC Ultra Inverse'
      |         title('IEC Ultra Inverse');
      |     case 'IEEE Moderately Inverse'
      |         title('IEEE Moderately Inverse');
      |     case 'IEEE Very Inverse'
      |         title('IEEE Very Inverse');
      |     case 'IEEE Extremely Inverse'
      |         title('IEEE Extremely Inverse');
      | end
      | ymax=10^ceil(log10(max(y)));
      | set(gca, 'XTick',[1:10 20]);
      | set(gca, 'YTick',[0 ymax/1000 ymax/500 ymax/200 ymax/100 ymax/50 ymax/20 ymax/10 ymax/5 ymax/2 ymax]);
      | xlim([0.9 30]);
      | ylim([0.01 ymax]);
      | xlabel(['Corriente multiplicada por Ipick-up(' num2str(PS*Vp) 'A)']);
      | ylabel('Tiempo de Operacion (Seg)');
      | grid on;
      | set(gca, 'color',[0.9608 0.9608 0.937]);
      | set(gca, 'gridcolor',[0 0.6902 0.3137]);
      mask Callback TMS3:
      | % Plotting IDMT Curve
      | clf('reset')
      | TMS = str2num(get_param(gcb,'TMS3'));
      | Vp = str2num(get_param(gcb,'Vp'));
      | PS=str2num(get_param(gcb,'PS3'));
      | k = str2num(get_param(gcb,'k3'));
      | alpha = str2num(get_param(gcb,'alpha3'));
      | B = str2num(get_param(gcb,'B3'));
      | Esc = str2num(get_param(gcb,'Esc3'));
      | Tins = str2num(get_param(gcb,'Tins3'));
      | I = [1.1:0.1:Esc];
      | I1=[Esc,Esc:0.1:30];
      | y=((k./((I.^alpha)-1))+B)*TMS;
      | Tin=[((k./((Esc.^alpha)-1))+B)*TMS,ones(1,length(I1)-1)*Tins];
      | loglog(I,y,'m');
      | hold on
      | loglog(I1,Tin,'m');
      | set(gcf, 'Position', [200 150 300 500]);
      | switch(get_param(gcb,'TCpopup3'))
      |     case 'IEC Standard Inverse'
      |         title('IEC Standard Inverse');
      |     case 'IEC Very Inverse'
      |         title('IEC Very Inverse');
      |     case 'IEC Long Time Inverse'
      |         title('IEC Long Time Inverse');
      |     case 'IEC Extremely Inverse'
      |         title('IEC Extremely Inverse');
      |      case 'IEC Ultra Inverse'
      |         title('IEC Ultra Inverse');
      |     case 'IEEE Moderately Inverse'
      |         title('IEEE Moderately Inverse');
      |     case 'IEEE Very Inverse'
      |         title('IEEE Very Inverse');
      |     case 'IEEE Extremely Inverse'
      |         title('IEEE Extremely Inverse');
      | end
      | ymax=10^ceil(log10(max(y)));
      | set(gca, 'XTick',[1:10 20]);
      | set(gca, 'YTick',[0 ymax/1000 ymax/500 ymax/200 ymax/100 ymax/50 ymax/20 ymax/10 ymax/5 ymax/2 ymax]);
      | xlim([0.9 30]);
      | ylim([0.01 ymax]);
      | xlabel(['Corriente multiplicada por Ipick-up(' num2str(PS*Vp) 'A)']);
      | ylabel('Tiempo de Operacion (Seg)');
      | grid on;
      | set(gca, 'color',[0.9608 0.9608 0.937]);
      | set(gca, 'gridcolor',[0 0.6902 0.3137]);
      mask Callback Tins3:
      | % Plotting IDMT Curve
      | clf('reset')
      | TMS = str2num(get_param(gcb,'TMS3'));
      | Vp = str2num(get_param(gcb,'Vp'));
      | PS=str2num(get_param(gcb,'PS3'));
      | k = str2num(get_param(gcb,'k3'));
      | alpha = str2num(get_param(gcb,'alpha3'));
      | B = str2num(get_param(gcb,'B3'));
      | Esc = str2num(get_param(gcb,'Esc3'));
      | Tins = str2num(get_param(gcb,'Tins3'));
      | I = [1.1:0.1:Esc];
      | I1=[Esc,Esc:0.1:30];
      | y=((k./((I.^alpha)-1))+B)*TMS;
      | Tin=[((k./((Esc.^alpha)-1))+B)*TMS,ones(1,length(I1)-1)*Tins];
      | loglog(I,y,'m');
      | hold on
      | loglog(I1,Tin,'m');
      | set(gcf, 'Position', [200 150 300 500]);
      | switch(get_param(gcb,'TCpopup3'))
      |     case 'IEC Standard Inverse'
      |         title('IEC Standard Inverse');
      |     case 'IEC Very Inverse'
      |         title('IEC Very Inverse');
      |     case 'IEC Long Time Inverse'
      |         title('IEC Long Time Inverse');
      |     case 'IEC Extremely Inverse'
      |         title('IEC Extremely Inverse');
      |      case 'IEC Ultra Inverse'
      |         title('IEC Ultra Inverse');
      |     case 'IEEE Moderately Inverse'
      |         title('IEEE Moderately Inverse');
      |     case 'IEEE Very Inverse'
      |         title('IEEE Very Inverse');
      |     case 'IEEE Extremely Inverse'
      |         title('IEEE Extremely Inverse');
      | end
      | ymax=10^ceil(log10(max(y)));
      | set(gca, 'XTick',[1:10 20]);
      | set(gca, 'YTick',[0 ymax/1000 ymax/500 ymax/200 ymax/100 ymax/50 ymax/20 ymax/10 ymax/5 ymax/2 ymax]);
      | xlim([0.9 30]);
      | ylim([0.01 ymax]);
      | xlabel(['Corriente multiplicada por Ipick-up(' num2str(PS*Vp) 'A)']);
      | ylabel('Tiempo de Operacion (Seg)');
      | grid on;
      | set(gca, 'color',[0.9608 0.9608 0.937]);
      | set(gca, 'gridcolor',[0 0.6902 0.3137]);
      mask Callback Esc3:
      | % Plotting IDMT Curve
      | clf('reset')
      | TMS = str2num(get_param(gcb,'TMS3'));
      | Vp = str2num(get_param(gcb,'Vp'));
      | PS=str2num(get_param(gcb,'PS3'));
      | k = str2num(get_param(gcb,'k3'));
      | alpha = str2num(get_param(gcb,'alpha3'));
      | B = str2num(get_param(gcb,'B3'));
      | Esc = str2num(get_param(gcb,'Esc3'));
      | Tins = str2num(get_param(gcb,'Tins3'));
      | I = [1.1:0.1:Esc];
      | I1=[Esc,Esc:0.1:30];
      | y=((k./((I.^alpha)-1))+B)*TMS;
      | Tin=[((k./((Esc.^alpha)-1))+B)*TMS,ones(1,length(I1)-1)*Tins];
      | loglog(I,y,'m');
      | hold on
      | loglog(I1,Tin,'m');
      | set(gcf, 'Position', [200 150 300 500]);
      | switch(get_param(gcb,'TCpopup3'))
      |     case 'IEC Standard Inverse'
      |         title('IEC Standard Inverse');
      |     case 'IEC Very Inverse'
      |         title('IEC Very Inverse');
      |     case 'IEC Long Time Inverse'
      |         title('IEC Long Time Inverse');
      |     case 'IEC Extremely Inverse'
      |         title('IEC Extremely Inverse');
      |      case 'IEC Ultra Inverse'
      |         title('IEC Ultra Inverse');
      |     case 'IEEE Moderately Inverse'
      |         title('IEEE Moderately Inverse');
      |     case 'IEEE Very Inverse'
      |         title('IEEE Very Inverse');
      |     case 'IEEE Extremely Inverse'
      |         title('IEEE Extremely Inverse');
      | end
      | ymax=10^ceil(log10(max(y)));
      | set(gca, 'XTick',[1:10 20]);
      | set(gca, 'YTick',[0 ymax/1000 ymax/500 ymax/200 ymax/100 ymax/50 ymax/20 ymax/10 ymax/5 ymax/2 ymax]);
      | xlim([0.9 30]);
      | ylim([0.01 ymax]);
      | xlabel(['Corriente multiplicada por Ipick-up(' num2str(PS*Vp) 'A)']);
      | ylabel('Tiempo de Operacion (Seg)');
      | grid on;
      | set(gca, 'color',[0.9608 0.9608 0.937]);
      | set(gca, 'gridcolor',[0 0.6902 0.3137]);
      mask DialogControl Container6 Prompt: Protecciones
      mask DialogControl Container8 Prompt: Topologia 1
      mask DialogControl Container9 Prompt: Proteccion 51
      mask DialogControl Container10 Prompt: Proteccion 50
      mask DialogControl Container8_copy Prompt: Topologia 2
      mask DialogControl Container9_copy Prompt: Proteccion 51
      mask DialogControl Container10_copy Prompt: Proteccion 50
      mask DialogControl Container8_copy_copy Prompt: Topologia 3
      mask DialogControl Container9_copy_copy Prompt: Proteccion 51
      mask DialogControl Container10_copy_copy Prompt: Proteccion 50
      mask DialogControl Container17 Prompt: Caracteristicas Trafo Corriente
      mask Display:
      | port_label('input',1,'D');
      | port_label('input',2,'I');
      | port_label('output',1,'S');
      | text(0.62, 0.5,'50', 'horizontalAlignment', 'center');
      | text(0.62, 0.3,'51', 'horizontalAlignment', 'center');
      | plot([0.08:0.01:0.32]+0.4,[0:0.01:0.24]*0+0.40);
      | plot(0.25*sin([0:pi/20:2*pi])+0.6,0.25*cos([0:pi/20:2*pi])+0.4);
      | %Linea Salida
      | plot([0.85:0.01:1],[0:0.01:0.15]*0+0.4);
      | %Linea Corriente
      | plot([0.2:0.01:0.35],[0:0.01:0.15]*0+0.4);
      | plot([0.1:0.01:0.2],[0:0.01:0.1]*0+0.15);
      | plot([0.1:0.01:0.35]*0+0.2,[0:0.01:0.25]+0.15);
      | %Linea tension
      | plot([0.15:0.01:0.6],[0:0.01:0.45]*0+0.7);
      | plot([0:0.01:0.05]*0+0.6,[0:0.01:0.05]+0.65);
  RB5 : Subsystem  mask(Proteccion de Sobrecorriente multitopologia){menu=3, TCpopup1=IEC Standard Inverse, k1=0.14, alpha1=0.02, B1=0, PS1=0.33, TMS1=0.529, Tins1=0.3, Esc1=7, TCpopup2=IEC Standard Inverse, k2=0.14, alpha2=0.02, B2=0, PS2=1.5, TMS2=0.2, Tins2=0.4, Esc2=6, TCpopup3=IEC Standard Inverse, k3=0.14, alpha3=0.02, B3=0, PS3=0.78, TMS3=0.25, Tins3=0.3, Esc3=8, Vp=200, Vs=5, F=60}
      mask prompts: menu "Numero de Topologias"; TCpopup1 "Caracteristica de Disparo"; k1 "k"; alpha1 "alpha"; B1 "B"; PS1 "Seteo disparo(PS)/Seteo inferior(I>)"; TMS1 "Multiplicador de Tiempo"; Tins1 "Tins"; Esc1 "Escala"; TCpopup2 "Caracteristica de Disparo"; k2 "k"; alpha2 "alpha"; B2 "B"; PS2 "Seteo disparo(PS)/Seteo inferior(I>)"; TMS2 "Multiplicador de tiempo"; Tins2 "Tins"; Esc2 "Escala"; TCpopup3 "Caracteristica de Disparo"; k3 "k"; alpha3 "alpha"; B3 "B"; PS3 "Seteo disparo(PS)/Seteo inferior(I>)"; TMS3 "Multiplicador de Tiempo"; Tins3 "Tins"; Esc3 "Escala"; Vp "Primario CT"; Vs "Secundario CT"; F "Frecuencia"
      mask help: Proteccion de Sobrecorriente con tres topologias internas controladas por una señal de control externa.
      mask init:
      | warning('off','Simulink:Masking:Invalid_Visible_Flag')
      mask TypeOptions menu: 1 | 2 | 3
      mask Callback menu:
      | h = getSimulinkBlockHandle(gcb);
      | menu1 = get_param(h,'menu');
      | if strcmp(menu1,num2str(1))
      |     set_param(h,'MaskVisibilities',{'on',...
      |         'on','on','on','on','on','on','on','on',...%proteccion 1 activa
      |         'off','off','off','off','off','off','off','off',...%proteccion 2 desactivada
      |         'off','off','off','off','off','off','off','off',...%proteccion 3 desactivada
      |         'on','on','on'});%Otros parametros activados
      |     Int=1;
      | elseif strcmp(menu1,num2str(2))
      |  set_param(h,'MaskVisibilities',{'on',...
      |         'on','on','on','on','on','on','on','on',...%proteccion 1 activa
      |         'on','on','on','on','on','on','on','on',...%proteccion 2 activa
      |         'off','off','off','off','off','off','off','off',...%proteccion 3 desactivada
      |         'on','on','on'});%Otros parametros activados
      |     Int=2;
      | else
      | set_param(h,'MaskVisibilities',{'on',...
      |         'on','on','on','on','on','on','on','on',...%proteccion 1 activa
      |         'on','on','on','on','on','on','on','on',...%proteccion 2 activa
      |         'on','on','on','on','on','on','on','on',...%proteccion 3 desactivada
      |         'on','on','on'});%Otros parametros activados
      |     Int=3;
      | end
      mask TypeOptions TCpopup1: IEC Standard Inverse | IEC Very Inverse | IEC Long Time Inverse | IEC Extremely Inverse | IEC Ultra Inverse | IEEE Moderately Inverse | IEEE Very Inverse | IEEE Extremely Inverse
      mask Callback TCpopup1:
      | switch(get_param(gcb,'TCpopup1'))
      |     case 'IEC Standard Inverse'
      |         set_param(gcb,'k1','0.14');
      |         set_param(gcb,'alpha1','0.02');
      |         set_param(gcb,'B1','0');
      |     case 'IEC Very Inverse'
      |         set_param(gcb,'k1','13.5');
      |         set_param(gcb,'alpha1','1');
      |         set_param(gcb,'B1','0');
      |     case 'IEC Long Time Inverse'
      |         set_param(gcb,'k1','120');
      |         set_param(gcb,'alpha1','1');
      |         set_param(gcb,'B1','0');
      |     case 'IEC Extremely Inverse'
      |         set_param(gcb,'k1','80');
      |         set_param(gcb,'alpha1','2');
      |         set_param(gcb,'B1','0');
      |     case 'IEC Ultra Inverse'
      |         set_param(gcb,'k1','315.2');
      |         set_param(gcb,'alpha1','2.5');
      |         set_param(gcb,'B1','0');
      |     case 'IEEE Moderately Inverse'
      |         set_param(gcb,'k1','0.0515');
      |         set_param(gcb,'alpha1','0.02');
      |         set_param(gcb,'B1','0.114');
      |     case 'IEEE Very Inverse'
      |         set_param(gcb,'k1','19.61');
      |         set_param(gcb,'alpha1','2');
      |         set_param(gcb,'B1','0.491');
      |     case 'IEEE Extremely Inverse'
      |         set_param(gcb,'k1','28.2');
      |         set_param(gcb,'alpha1','2');
      |         set_param(gcb,'B1','0.1217');
      | end
      | % Plotting IDMT Curve
      | clf('reset')
      | TMS = str2num(get_param(gcb,'TMS1'));
      | Vp = str2num(get_param(gcb,'Vp'));
      | PS=str2num(get_param(gcb,'PS1'));
      | k = str2num(get_param(gcb,'k1'));
      | alpha = str2num(get_param(gcb,'alpha1'));
      | B = str2num(get_param(gcb,'B1'));
      | Esc = str2num(get_param(gcb,'Esc1'));
      | Tins = str2num(get_param(gcb,'Tins1'));
      | I = [1.1:0.1:Esc];
      | I1=[Esc,Esc:0.1:30];
      | y=((k./((I.^alpha)-1))+B)*TMS;
      | Tin=[((k./((Esc.^alpha)-1))+B)*TMS,ones(1,length(I1)-1)*Tins];
      | loglog(I,y,'b');
      | hold on
      | loglog(I1,Tin,'b');
      | set(gcf, 'Position', [200 150 300 500]);
      | switch(get_param(gcb,'TCpopup1'))
      |     case 'IEC Standard Inverse'
      |         title('IEC Standard Inverse');
      |     case 'IEC Very Inverse'
      |         title('IEC Very Inverse');
      |     case 'IEC Long Time Inverse'
      |         title('IEC Long Time Inverse');
      |     case 'IEC Extremely Inverse'
      |         title('IEC Extremely Inverse');
      |      case 'IEC Ultra Inverse'
      |         title('IEC Ultra Inverse');
      |     case 'IEEE Moderately Inverse'
      |         title('IEEE Moderately Inverse');
      |     case 'IEEE Very Inverse'
      |         title('IEEE Very Inverse');
      |     case 'IEEE Extremely Inverse'
      |         title('IEEE Extremely Inverse');
      | end
      | ymax=10^ceil(log10(max(y)));
      | set(gca, 'XTick',[1:10 20]);
      | set(gca, 'YTick',[0 ymax/1000 ymax/500 ymax/200 ymax/100 ymax/50 ymax/20 ymax/10 ymax/5 ymax/2 ymax]);
      | xlim([0.9 30]);
      | ylim([0.01 ymax]);
      | xlabel(['Corriente multiplicada por Ipick-up(' num2str(PS*Vp) 'A)']);
      | ylabel('Tiempo de Operacion (Seg)');
      | grid on;
      | set(gca, 'color',[0.9608 0.9608 0.937]);
      | set(gca, 'gridcolor',[0 0.6902 0.3137]);
      mask Callback PS1:
      | % Plotting IDMT Curve
      | clf('reset')
      | TMS = str2num(get_param(gcb,'TMS1'));
      | Vp = str2num(get_param(gcb,'Vp'));
      | PS=str2num(get_param(gcb,'PS1'));
      | k = str2num(get_param(gcb,'k1'));
      | alpha = str2num(get_param(gcb,'alpha1'));
      | B = str2num(get_param(gcb,'B1'));
      | Esc = str2num(get_param(gcb,'Esc1'));
      | Tins = str2num(get_param(gcb,'Tins1'));
      | I = [1.1:0.1:Esc];
      | I1=[Esc,Esc:0.1:30];
      | y=((k./((I.^alpha)-1))+B)*TMS;
      | Tin=[((k./((Esc.^alpha)-1))+B)*TMS,ones(1,length(I1)-1)*Tins];
      | loglog(I,y,'b');
      | hold on
      | loglog(I1,Tin,'b');
      | set(gcf, 'Position', [200 150 300 500]);
      | switch(get_param(gcb,'TCpopup1'))
      |     case 'IEC Standard Inverse'
      |         title('IEC Standard Inverse');
      |     case 'IEC Very Inverse'
      |         title('IEC Very Inverse');
      |     case 'IEC Long Time Inverse'
      |         title('IEC Long Time Inverse');
      |     case 'IEC Extremely Inverse'
      |         title('IEC Extremely Inverse');
      |      case 'IEC Ultra Inverse'
      |         title('IEC Ultra Inverse');
      |     case 'IEEE Moderately Inverse'
      |         title('IEEE Moderately Inverse');
      |     case 'IEEE Very Inverse'
      |         title('IEEE Very Inverse');
      |     case 'IEEE Extremely Inverse'
      |         title('IEEE Extremely Inverse');
      | end
      | ymax=10^ceil(log10(max(y)));
      | set(gca, 'XTick',[1:10 20]);
      | set(gca, 'YTick',[0 ymax/1000 ymax/500 ymax/200 ymax/100 ymax/50 ymax/20 ymax/10 ymax/5 ymax/2 ymax]);
      | xlim([0.9 30]);
      | ylim([0.01 ymax]);
      | xlabel(['Corriente multiplicada por Ipick-up(' num2str(PS*Vp) 'A)']);
      | ylabel('Tiempo de Operacion (Seg)');
      | grid on;
      | set(gca, 'color',[0.9608 0.9608 0.937]);
      | set(gca, 'gridcolor',[0 0.6902 0.3137]);
      mask Callback TMS1:
      | % Plotting IDMT Curve
      | clf('reset')
      | TMS = str2num(get_param(gcb,'TMS1'));
      | Vp = str2num(get_param(gcb,'Vp'));
      | PS=str2num(get_param(gcb,'PS1'));
      | k = str2num(get_param(gcb,'k1'));
      | alpha = str2num(get_param(gcb,'alpha1'));
      | B = str2num(get_param(gcb,'B1'));
      | Esc = str2num(get_param(gcb,'Esc1'));
      | Tins = str2num(get_param(gcb,'Tins1'));
      | I = [1.1:0.1:Esc];
      | I1=[Esc,Esc:0.1:30];
      | y=((k./((I.^alpha)-1))+B)*TMS;
      | Tin=[((k./((Esc.^alpha)-1))+B)*TMS,ones(1,length(I1)-1)*Tins];
      | loglog(I,y,'b');
      | hold on
      | loglog(I1,Tin,'b');
      | set(gcf, 'Position', [200 150 300 500]);
      | switch(get_param(gcb,'TCpopup1'))
      |     case 'IEC Standard Inverse'
      |         title('IEC Standard Inverse');
      |     case 'IEC Very Inverse'
      |         title('IEC Very Inverse');
      |     case 'IEC Long Time Inverse'
      |         title('IEC Long Time Inverse');
      |     case 'IEC Extremely Inverse'
      |         title('IEC Extremely Inverse');
      |      case 'IEC Ultra Inverse'
      |         title('IEC Ultra Inverse');
      |     case 'IEEE Moderately Inverse'
      |         title('IEEE Moderately Inverse');
      |     case 'IEEE Very Inverse'
      |         title('IEEE Very Inverse');
      |     case 'IEEE Extremely Inverse'
      |         title('IEEE Extremely Inverse');
      | end
      | ymax=10^ceil(log10(max(y)));
      | set(gca, 'XTick',[1:10 20]);
      | set(gca, 'YTick',[0 ymax/1000 ymax/500 ymax/200 ymax/100 ymax/50 ymax/20 ymax/10 ymax/5 ymax/2 ymax]);
      | xlim([0.9 30]);
      | ylim([0.01 ymax]);
      | xlabel(['Corriente multiplicada por Ipick-up(' num2str(PS*Vp) 'A)']);
      | ylabel('Tiempo de Operacion (Seg)');
      | grid on;
      | set(gca, 'color',[0.9608 0.9608 0.937]);
      | set(gca, 'gridcolor',[0 0.6902 0.3137]);
      mask Callback Tins1:
      | % Plotting IDMT Curve
      | clf('reset')
      | TMS = str2num(get_param(gcb,'TMS1'));
      | Vp = str2num(get_param(gcb,'Vp'));
      | PS=str2num(get_param(gcb,'PS1'));
      | k = str2num(get_param(gcb,'k1'));
      | alpha = str2num(get_param(gcb,'alpha1'));
      | B = str2num(get_param(gcb,'B1'));
      | Esc = str2num(get_param(gcb,'Esc1'));
      | Tins = str2num(get_param(gcb,'Tins1'));
      | I = [1.1:0.1:Esc];
      | I1=[Esc,Esc:0.1:30];
      | y=((k./((I.^alpha)-1))+B)*TMS;
      | Tin=[((k./((Esc.^alpha)-1))+B)*TMS,ones(1,length(I1)-1)*Tins];
      | loglog(I,y,'b');
      | hold on
      | loglog(I1,Tin,'b');
      | set(gcf, 'Position', [200 150 300 500]);
      | switch(get_param(gcb,'TCpopup1'))
      |     case 'IEC Standard Inverse'
      |         title('IEC Standard Inverse');
      |     case 'IEC Very Inverse'
      |         title('IEC Very Inverse');
      |     case 'IEC Long Time Inverse'
      |         title('IEC Long Time Inverse');
      |     case 'IEC Extremely Inverse'
      |         title('IEC Extremely Inverse');
      |      case 'IEC Ultra Inverse'
      |         title('IEC Ultra Inverse');
      |     case 'IEEE Moderately Inverse'
      |         title('IEEE Moderately Inverse');
      |     case 'IEEE Very Inverse'
      |         title('IEEE Very Inverse');
      |     case 'IEEE Extremely Inverse'
      |         title('IEEE Extremely Inverse');
      | end
      | ymax=10^ceil(log10(max(y)));
      | set(gca, 'XTick',[1:10 20]);
      | set(gca, 'YTick',[0 ymax/1000 ymax/500 ymax/200 ymax/100 ymax/50 ymax/20 ymax/10 ymax/5 ymax/2 ymax]);
      | xlim([0.9 30]);
      | ylim([0.01 ymax]);
      | xlabel(['Corriente multiplicada por Ipick-up(' num2str(PS*Vp) 'A)']);
      | ylabel('Tiempo de Operacion (Seg)');
      | grid on;
      | set(gca, 'color',[0.9608 0.9608 0.937]);
      | set(gca, 'gridcolor',[0 0.6902 0.3137]);
      mask Callback Esc1:
      | % Plotting IDMT Curve
      | clf('reset')
      | TMS = str2num(get_param(gcb,'TMS1'));
      | Vp = str2num(get_param(gcb,'Vp'));
      | PS=str2num(get_param(gcb,'PS1'));
      | k = str2num(get_param(gcb,'k1'));
      | alpha = str2num(get_param(gcb,'alpha1'));
      | B = str2num(get_param(gcb,'B1'));
      | Esc = str2num(get_param(gcb,'Esc1'));
      | Tins = str2num(get_param(gcb,'Tins1'));
      | I = [1.1:0.1:Esc];
      | I1=[Esc,Esc:0.1:30];
      | y=((k./((I.^alpha)-1))+B)*TMS;
      | Tin=[((k./((Esc.^alpha)-1))+B)*TMS,ones(1,length(I1)-1)*Tins];
      | loglog(I,y,'b');
      | hold on
      | loglog(I1,Tin,'b');
      | set(gcf, 'Position', [200 150 300 500]);
      | switch(get_param(gcb,'TCpopup1'))
      |     case 'IEC Standard Inverse'
      |         title('IEC Standard Inverse');
      |     case 'IEC Very Inverse'
      |         title('IEC Very Inverse');
      |     case 'IEC Long Time Inverse'
      |         title('IEC Long Time Inverse');
      |     case 'IEC Extremely Inverse'
      |         title('IEC Extremely Inverse');
      |      case 'IEC Ultra Inverse'
      |         title('IEC Ultra Inverse');
      |     case 'IEEE Moderately Inverse'
      |         title('IEEE Moderately Inverse');
      |     case 'IEEE Very Inverse'
      |         title('IEEE Very Inverse');
      |     case 'IEEE Extremely Inverse'
      |         title('IEEE Extremely Inverse');
      | end
      | ymax=10^ceil(log10(max(y)));
      | set(gca, 'XTick',[1:10 20]);
      | set(gca, 'YTick',[0 ymax/1000 ymax/500 ymax/200 ymax/100 ymax/50 ymax/20 ymax/10 ymax/5 ymax/2 ymax]);
      | xlim([0.9 30]);
      | ylim([0.01 ymax]);
      | xlabel(['Corriente multiplicada por Ipick-up(' num2str(PS*Vp) 'A)']);
      | ylabel('Tiempo de Operacion (Seg)');
      | grid on;
      | set(gca, 'color',[0.9608 0.9608 0.937]);
      | set(gca, 'gridcolor',[0 0.6902 0.3137]);
      mask TypeOptions TCpopup2: IEC Standard Inverse | IEC Very Inverse | IEC Long Time Inverse | IEC Extremely Inverse | IEC Ultra Inverse | IEEE Moderately Inverse | IEEE Very Inverse | IEEE Extremely Inverse
      mask Callback TCpopup2:
      | switch(get_param(gcb,'TCpopup2'))
      |     case 'IEC Standard Inverse'
      |         set_param(gcb,'k2','0.14');
      |         set_param(gcb,'alpha2','0.02');
      |         set_param(gcb,'B2','0');
      |     case 'IEC Very Inverse'
      |         set_param(gcb,'k2','13.5');
      |         set_param(gcb,'alpha2','1');
      |         set_param(gcb,'B2','0');
      |     case 'IEC Long Time Inverse'
      |         set_param(gcb,'k2','120');
      |         set_param(gcb,'alpha2','1');
      |         set_param(gcb,'B2','0');
      |     case 'IEC Extremely Inverse'
      |         set_param(gcb,'k2','80');
      |         set_param(gcb,'alpha2','2');
      |         set_param(gcb,'B2','0');
      |     case 'IEC Ultra Inverse'
      |         set_param(gcb,'k2','315.2');
      |         set_param(gcb,'alpha2','2.5');
      |         set_param(gcb,'B2','0');
      |     case 'IEEE Moderately Inverse'
      |         set_param(gcb,'k2','0.0515');
      |         set_param(gcb,'alpha2','0.02');
      |         set_param(gcb,'B2','0.114');
      |     case 'IEEE Very Inverse'
      |         set_param(gcb,'k2','19.61');
      |         set_param(gcb,'alpha2','2');
      |         set_param(gcb,'B2','0.491');
      |     case 'IEEE Extremely Inverse'
      |         set_param(gcb,'k2','28.2');
      |         set_param(gcb,'alpha2','2');
      |         set_param(gcb,'B2','0.1217');
      | end
      | % Plotting IDMT Curve
      | clf('reset')
      | TMS = str2num(get_param(gcb,'TMS2'));
      | Vp = str2num(get_param(gcb,'Vp'));
      | PS=str2num(get_param(gcb,'PS2'));
      | k = str2num(get_param(gcb,'k2'));
      | alpha = str2num(get_param(gcb,'alpha2'));
      | B = str2num(get_param(gcb,'B2'));
      | Esc = str2num(get_param(gcb,'Esc2'));
      | Tins = str2num(get_param(gcb,'Tins2'));
      | I = [1.1:0.1:Esc];
      | I1=[Esc,Esc:0.1:30];
      | y=((k./((I.^alpha)-1))+B)*TMS;
      | Tin=[((k./((Esc.^alpha)-1))+B)*TMS,ones(1,length(I1)-1)*Tins];
      | loglog(I,y,'r');
      | hold on
      | loglog(I1,Tin,'r');
      | set(gcf, 'Position', [200 150 300 500]);
      | switch(get_param(gcb,'TCpopup2'))
      |     case 'IEC Standard Inverse'
      |         title('IEC Standard Inverse');
      |     case 'IEC Very Inverse'
      |         title('IEC Very Inverse');
      |     case 'IEC Long Time Inverse'
      |         title('IEC Long Time Inverse');
      |     case 'IEC Extremely Inverse'
      |         title('IEC Extremely Inverse');
      |      case 'IEC Ultra Inverse'
      |         title('IEC Ultra Inverse');
      |     case 'IEEE Moderately Inverse'
      |         title('IEEE Moderately Inverse');
      |     case 'IEEE Very Inverse'
      |         title('IEEE Very Inverse');
      |     case 'IEEE Extremely Inverse'
      |         title('IEEE Extremely Inverse');
      | end
      | ymax=10^ceil(log10(max(y)));
      | set(gca, 'XTick',[1:10 20]);
      | set(gca, 'YTick',[0 ymax/1000 ymax/500 ymax/200 ymax/100 ymax/50 ymax/20 ymax/10 ymax/5 ymax/2 ymax]);
      | xlim([0.9 30]);
      | ylim([0.01 ymax]);
      | xlabel(['Corriente multiplicada por Ipick-up(' num2str(PS*Vp) 'A)']);
      | ylabel('Tiempo de Operacion (Seg)');
      | grid on;
      | set(gca, 'color',[0.9608 0.9608 0.937]);
      | set(gca, 'gridcolor',[0 0.6902 0.3137]);
      mask Callback PS2:
      | % Plotting IDMT Curve
      | clf('reset')
      | TMS = str2num(get_param(gcb,'TMS2'));
      | Vp = str2num(get_param(gcb,'Vp'));
      | PS=str2num(get_param(gcb,'PS2'));
      | k = str2num(get_param(gcb,'k2'));
      | alpha = str2num(get_param(gcb,'alpha2'));
      | B = str2num(get_param(gcb,'B2'));
      | Esc = str2num(get_param(gcb,'Esc2'));
      | Tins = str2num(get_param(gcb,'Tins2'));
      | I = [1.1:0.1:Esc];
      | I1=[Esc,Esc:0.1:30];
      | y=((k./((I.^alpha)-1))+B)*TMS;
      | Tin=[((k./((Esc.^alpha)-1))+B)*TMS,ones(1,length(I1)-1)*Tins];
      | loglog(I,y,'r');
      | hold on
      | loglog(I1,Tin,'r');
      | set(gcf, 'Position', [200 150 300 500]);
      | switch(get_param(gcb,'TCpopup2'))
      |     case 'IEC Standard Inverse'
      |         title('IEC Standard Inverse');
      |     case 'IEC Very Inverse'
      |         title('IEC Very Inverse');
      |     case 'IEC Long Time Inverse'
      |         title('IEC Long Time Inverse');
      |     case 'IEC Extremely Inverse'
      |         title('IEC Extremely Inverse');
      |      case 'IEC Ultra Inverse'
      |         title('IEC Ultra Inverse');
      |     case 'IEEE Moderately Inverse'
      |         title('IEEE Moderately Inverse');
      |     case 'IEEE Very Inverse'
      |         title('IEEE Very Inverse');
      |     case 'IEEE Extremely Inverse'
      |         title('IEEE Extremely Inverse');
      | end
      | ymax=10^ceil(log10(max(y)));
      | set(gca, 'XTick',[1:10 20]);
      | set(gca, 'YTick',[0 ymax/1000 ymax/500 ymax/200 ymax/100 ymax/50 ymax/20 ymax/10 ymax/5 ymax/2 ymax]);
      | xlim([0.9 30]);
      | ylim([0.01 ymax]);
      | xlabel(['Corriente multiplicada por Ipick-up(' num2str(PS*Vp) 'A)']);
      | ylabel('Tiempo de Operacion (Seg)');
      | grid on;
      | set(gca, 'color',[0.9608 0.9608 0.937]);
      | set(gca, 'gridcolor',[0 0.6902 0.3137]);
      mask Callback TMS2:
      | % Plotting IDMT Curve
      | clf('reset')
      | TMS = str2num(get_param(gcb,'TMS2'));
      | Vp = str2num(get_param(gcb,'Vp'));
      | PS=str2num(get_param(gcb,'PS2'));
      | k = str2num(get_param(gcb,'k2'));
      | alpha = str2num(get_param(gcb,'alpha2'));
      | B = str2num(get_param(gcb,'B2'));
      | Esc = str2num(get_param(gcb,'Esc2'));
      | Tins = str2num(get_param(gcb,'Tins2'));
      | I = [1.1:0.1:Esc];
      | I1=[Esc,Esc:0.1:30];
      | y=((k./((I.^alpha)-1))+B)*TMS;
      | Tin=[((k./((Esc.^alpha)-1))+B)*TMS,ones(1,length(I1)-1)*Tins];
      | loglog(I,y,'r');
      | hold on
      | loglog(I1,Tin,'r');
      | set(gcf, 'Position', [200 150 300 500]);
      | switch(get_param(gcb,'TCpopup2'))
      |     case 'IEC Standard Inverse'
      |         title('IEC Standard Inverse');
      |     case 'IEC Very Inverse'
      |         title('IEC Very Inverse');
      |     case 'IEC Long Time Inverse'
      |         title('IEC Long Time Inverse');
      |     case 'IEC Extremely Inverse'
      |         title('IEC Extremely Inverse');
      |      case 'IEC Ultra Inverse'
      |         title('IEC Ultra Inverse');
      |     case 'IEEE Moderately Inverse'
      |         title('IEEE Moderately Inverse');
      |     case 'IEEE Very Inverse'
      |         title('IEEE Very Inverse');
      |     case 'IEEE Extremely Inverse'
      |         title('IEEE Extremely Inverse');
      | end
      | ymax=10^ceil(log10(max(y)));
      | set(gca, 'XTick',[1:10 20]);
      | set(gca, 'YTick',[0 ymax/1000 ymax/500 ymax/200 ymax/100 ymax/50 ymax/20 ymax/10 ymax/5 ymax/2 ymax]);
      | xlim([0.9 30]);
      | ylim([0.01 ymax]);
      | xlabel(['Corriente multiplicada por Ipick-up(' num2str(PS*Vp) 'A)']);
      | ylabel('Tiempo de Operacion (Seg)');
      | grid on;
      | set(gca, 'color',[0.9608 0.9608 0.937]);
      | set(gca, 'gridcolor',[0 0.6902 0.3137]);
      mask Callback Tins2:
      | % Plotting IDMT Curve
      | clf('reset')
      | TMS = str2num(get_param(gcb,'TMS2'));
      | Vp = str2num(get_param(gcb,'Vp'));
      | PS=str2num(get_param(gcb,'PS2'));
      | k = str2num(get_param(gcb,'k2'));
      | alpha = str2num(get_param(gcb,'alpha2'));
      | B = str2num(get_param(gcb,'B2'));
      | Esc = str2num(get_param(gcb,'Esc2'));
      | Tins = str2num(get_param(gcb,'Tins2'));
      | I = [1.1:0.1:Esc];
      | I1=[Esc,Esc:0.1:30];
      | y=((k./((I.^alpha)-1))+B)*TMS;
      | Tin=[((k./((Esc.^alpha)-1))+B)*TMS,ones(1,length(I1)-1)*Tins];
      | loglog(I,y,'r');
      | hold on
      | loglog(I1,Tin,'r');
      | set(gcf, 'Position', [200 150 300 500]);
      | switch(get_param(gcb,'TCpopup2'))
      |     case 'IEC Standard Inverse'
      |         title('IEC Standard Inverse');
      |     case 'IEC Very Inverse'
      |         title('IEC Very Inverse');
      |     case 'IEC Long Time Inverse'
      |         title('IEC Long Time Inverse');
      |     case 'IEC Extremely Inverse'
      |         title('IEC Extremely Inverse');
      |      case 'IEC Ultra Inverse'
      |         title('IEC Ultra Inverse');
      |     case 'IEEE Moderately Inverse'
      |         title('IEEE Moderately Inverse');
      |     case 'IEEE Very Inverse'
      |         title('IEEE Very Inverse');
      |     case 'IEEE Extremely Inverse'
      |         title('IEEE Extremely Inverse');
      | end
      | ymax=10^ceil(log10(max(y)));
      | set(gca, 'XTick',[1:10 20]);
      | set(gca, 'YTick',[0 ymax/1000 ymax/500 ymax/200 ymax/100 ymax/50 ymax/20 ymax/10 ymax/5 ymax/2 ymax]);
      | xlim([0.9 30]);
      | ylim([0.01 ymax]);
      | xlabel(['Corriente multiplicada por Ipick-up(' num2str(PS*Vp) 'A)']);
      | ylabel('Tiempo de Operacion (Seg)');
      | grid on;
      | set(gca, 'color',[0.9608 0.9608 0.937]);
      | set(gca, 'gridcolor',[0 0.6902 0.3137]);
      mask Callback Esc2:
      | % Plotting IDMT Curve
      | clf('reset')
      | TMS = str2num(get_param(gcb,'TMS2'));
      | Vp = str2num(get_param(gcb,'Vp'));
      | PS=str2num(get_param(gcb,'PS2'));
      | k = str2num(get_param(gcb,'k2'));
      | alpha = str2num(get_param(gcb,'alpha2'));
      | B = str2num(get_param(gcb,'B2'));
      | Esc = str2num(get_param(gcb,'Esc2'));
      | Tins = str2num(get_param(gcb,'Tins2'));
      | I = [1.1:0.1:Esc];
      | I1=[Esc,Esc:0.1:30];
      | y=((k./((I.^alpha)-1))+B)*TMS;
      | Tin=[((k./((Esc.^alpha)-1))+B)*TMS,ones(1,length(I1)-1)*Tins];
      | loglog(I,y,'r');
      | hold on
      | loglog(I1,Tin,'r');
      | set(gcf, 'Position', [200 150 300 500]);
      | switch(get_param(gcb,'TCpopup2'))
      |     case 'IEC Standard Inverse'
      |         title('IEC Standard Inverse');
      |     case 'IEC Very Inverse'
      |         title('IEC Very Inverse');
      |     case 'IEC Long Time Inverse'
      |         title('IEC Long Time Inverse');
      |     case 'IEC Extremely Inverse'
      |         title('IEC Extremely Inverse');
      |      case 'IEC Ultra Inverse'
      |         title('IEC Ultra Inverse');
      |     case 'IEEE Moderately Inverse'
      |         title('IEEE Moderately Inverse');
      |     case 'IEEE Very Inverse'
      |         title('IEEE Very Inverse');
      |     case 'IEEE Extremely Inverse'
      |         title('IEEE Extremely Inverse');
      | end
      | ymax=10^ceil(log10(max(y)));
      | set(gca, 'XTick',[1:10 20]);
      | set(gca, 'YTick',[0 ymax/1000 ymax/500 ymax/200 ymax/100 ymax/50 ymax/20 ymax/10 ymax/5 ymax/2 ymax]);
      | xlim([0.9 30]);
      | ylim([0.01 ymax]);
      | xlabel(['Corriente multiplicada por Ipick-up(' num2str(PS*Vp) 'A)']);
      | ylabel('Tiempo de Operacion (Seg)');
      | grid on;
      | set(gca, 'color',[0.9608 0.9608 0.937]);
      | set(gca, 'gridcolor',[0 0.6902 0.3137]);
      mask TypeOptions TCpopup3: IEC Standard Inverse | IEC Very Inverse | IEC Long Time Inverse | IEC Extremely Inverse | IEC Ultra Inverse | IEEE Moderately Inverse | IEEE Very Inverse | IEEE Extremely Inverse
      mask Callback TCpopup3:
      | switch(get_param(gcb,'TCpopup3'))
      |     case 'IEC Standard Inverse'
      |         set_param(gcb,'k3','0.14');
      |         set_param(gcb,'alpha3','0.02');
      |         set_param(gcb,'B3','0');
      |     case 'IEC Very Inverse'
      |         set_param(gcb,'k3','13.5');
      |         set_param(gcb,'alpha3','1');
      |         set_param(gcb,'B3','0');
      |     case 'IEC Long Time Inverse'
      |         set_param(gcb,'k3','120');
      |         set_param(gcb,'alpha3','1');
      |         set_param(gcb,'B3','0');
      |     case 'IEC Extremely Inverse'
      |         set_param(gcb,'k3','80');
      |         set_param(gcb,'alpha3','2');
      |         set_param(gcb,'B3','0');
      |     case 'IEC Ultra Inverse'
      |         set_param(gcb,'k3','315.2');
      |         set_param(gcb,'alpha3','2.5');
      |         set_param(gcb,'B3','0');
      |     case 'IEEE Moderately Inverse'
      |         set_param(gcb,'k3','0.0515');
      |         set_param(gcb,'alpha3','0.02');
      |         set_param(gcb,'B3','0.114');
      |     case 'IEEE Very Inverse'
      |         set_param(gcb,'k3','19.61');
      |         set_param(gcb,'alpha3','2');
      |         set_param(gcb,'B3','0.491');
      |     case 'IEEE Extremely Inverse'
      |         set_param(gcb,'k3','28.2');
      |         set_param(gcb,'alpha3','2');
      |         set_param(gcb,'B3','0.1217');
      | end
      | % Plotting IDMT Curve
      | clf('reset')
      | TMS = str2num(get_param(gcb,'TMS3'));
      | Vp = str2num(get_param(gcb,'Vp'));
      | PS=str2num(get_param(gcb,'PS3'));
      | k = str2num(get_param(gcb,'k3'));
      | alpha = str2num(get_param(gcb,'alpha3'));
      | B = str2num(get_param(gcb,'B3'));
      | Esc = str2num(get_param(gcb,'Esc3'));
      | Tins = str2num(get_param(gcb,'Tins3'));
      | I = [1.1:0.1:Esc];
      | I1=[Esc,Esc:0.1:30];
      | y=((k./((I.^alpha)-1))+B)*TMS;
      | Tin=[((k./((Esc.^alpha)-1))+B)*TMS,ones(1,length(I1)-1)*Tins];
      | loglog(I,y,'m');
      | hold on
      | loglog(I1,Tin,'m');
      | set(gcf, 'Position', [200 150 300 500]);
      | switch(get_param(gcb,'TCpopup3'))
      |     case 'IEC Standard Inverse'
      |         title('IEC Standard Inverse');
      |     case 'IEC Very Inverse'
      |         title('IEC Very Inverse');
      |     case 'IEC Long Time Inverse'
      |         title('IEC Long Time Inverse');
      |     case 'IEC Extremely Inverse'
      |         title('IEC Extremely Inverse');
      |      case 'IEC Ultra Inverse'
      |         title('IEC Ultra Inverse');
      |     case 'IEEE Moderately Inverse'
      |         title('IEEE Moderately Inverse');
      |     case 'IEEE Very Inverse'
      |         title('IEEE Very Inverse');
      |     case 'IEEE Extremely Inverse'
      |         title('IEEE Extremely Inverse');
      | end
      | ymax=10^ceil(log10(max(y)));
      | set(gca, 'XTick',[1:10 20]);
      | set(gca, 'YTick',[0 ymax/1000 ymax/500 ymax/200 ymax/100 ymax/50 ymax/20 ymax/10 ymax/5 ymax/2 ymax]);
      | xlim([0.9 30]);
      | ylim([0.01 ymax]);
      | xlabel(['Corriente multiplicada por Ipick-up(' num2str(PS*Vp) 'A)']);
      | ylabel('Tiempo de Operacion (Seg)');
      | grid on;
      | set(gca, 'color',[0.9608 0.9608 0.937]);
      | set(gca, 'gridcolor',[0 0.6902 0.3137]);
      mask Callback PS3:
      | % Plotting IDMT Curve
      | clf('reset')
      | TMS = str2num(get_param(gcb,'TMS3'));
      | Vp = str2num(get_param(gcb,'Vp'));
      | PS=str2num(get_param(gcb,'PS3'));
      | k = str2num(get_param(gcb,'k3'));
      | alpha = str2num(get_param(gcb,'alpha3'));
      | B = str2num(get_param(gcb,'B3'));
      | Esc = str2num(get_param(gcb,'Esc3'));
      | Tins = str2num(get_param(gcb,'Tins3'));
      | I = [1.1:0.1:Esc];
      | I1=[Esc,Esc:0.1:30];
      | y=((k./((I.^alpha)-1))+B)*TMS;
      | Tin=[((k./((Esc.^alpha)-1))+B)*TMS,ones(1,length(I1)-1)*Tins];
      | loglog(I,y,'m');
      | hold on
      | loglog(I1,Tin,'m');
      | set(gcf, 'Position', [200 150 300 500]);
      | switch(get_param(gcb,'TCpopup3'))
      |     case 'IEC Standard Inverse'
      |         title('IEC Standard Inverse');
      |     case 'IEC Very Inverse'
      |         title('IEC Very Inverse');
      |     case 'IEC Long Time Inverse'
      |         title('IEC Long Time Inverse');
      |     case 'IEC Extremely Inverse'
      |         title('IEC Extremely Inverse');
      |      case 'IEC Ultra Inverse'
      |         title('IEC Ultra Inverse');
      |     case 'IEEE Moderately Inverse'
      |         title('IEEE Moderately Inverse');
      |     case 'IEEE Very Inverse'
      |         title('IEEE Very Inverse');
      |     case 'IEEE Extremely Inverse'
      |         title('IEEE Extremely Inverse');
      | end
      | ymax=10^ceil(log10(max(y)));
      | set(gca, 'XTick',[1:10 20]);
      | set(gca, 'YTick',[0 ymax/1000 ymax/500 ymax/200 ymax/100 ymax/50 ymax/20 ymax/10 ymax/5 ymax/2 ymax]);
      | xlim([0.9 30]);
      | ylim([0.01 ymax]);
      | xlabel(['Corriente multiplicada por Ipick-up(' num2str(PS*Vp) 'A)']);
      | ylabel('Tiempo de Operacion (Seg)');
      | grid on;
      | set(gca, 'color',[0.9608 0.9608 0.937]);
      | set(gca, 'gridcolor',[0 0.6902 0.3137]);
      mask Callback TMS3:
      | % Plotting IDMT Curve
      | clf('reset')
      | TMS = str2num(get_param(gcb,'TMS3'));
      | Vp = str2num(get_param(gcb,'Vp'));
      | PS=str2num(get_param(gcb,'PS3'));
      | k = str2num(get_param(gcb,'k3'));
      | alpha = str2num(get_param(gcb,'alpha3'));
      | B = str2num(get_param(gcb,'B3'));
      | Esc = str2num(get_param(gcb,'Esc3'));
      | Tins = str2num(get_param(gcb,'Tins3'));
      | I = [1.1:0.1:Esc];
      | I1=[Esc,Esc:0.1:30];
      | y=((k./((I.^alpha)-1))+B)*TMS;
      | Tin=[((k./((Esc.^alpha)-1))+B)*TMS,ones(1,length(I1)-1)*Tins];
      | loglog(I,y,'m');
      | hold on
      | loglog(I1,Tin,'m');
      | set(gcf, 'Position', [200 150 300 500]);
      | switch(get_param(gcb,'TCpopup3'))
      |     case 'IEC Standard Inverse'
      |         title('IEC Standard Inverse');
      |     case 'IEC Very Inverse'
      |         title('IEC Very Inverse');
      |     case 'IEC Long Time Inverse'
      |         title('IEC Long Time Inverse');
      |     case 'IEC Extremely Inverse'
      |         title('IEC Extremely Inverse');
      |      case 'IEC Ultra Inverse'
      |         title('IEC Ultra Inverse');
      |     case 'IEEE Moderately Inverse'
      |         title('IEEE Moderately Inverse');
      |     case 'IEEE Very Inverse'
      |         title('IEEE Very Inverse');
      |     case 'IEEE Extremely Inverse'
      |         title('IEEE Extremely Inverse');
      | end
      | ymax=10^ceil(log10(max(y)));
      | set(gca, 'XTick',[1:10 20]);
      | set(gca, 'YTick',[0 ymax/1000 ymax/500 ymax/200 ymax/100 ymax/50 ymax/20 ymax/10 ymax/5 ymax/2 ymax]);
      | xlim([0.9 30]);
      | ylim([0.01 ymax]);
      | xlabel(['Corriente multiplicada por Ipick-up(' num2str(PS*Vp) 'A)']);
      | ylabel('Tiempo de Operacion (Seg)');
      | grid on;
      | set(gca, 'color',[0.9608 0.9608 0.937]);
      | set(gca, 'gridcolor',[0 0.6902 0.3137]);
      mask Callback Tins3:
      | % Plotting IDMT Curve
      | clf('reset')
      | TMS = str2num(get_param(gcb,'TMS3'));
      | Vp = str2num(get_param(gcb,'Vp'));
      | PS=str2num(get_param(gcb,'PS3'));
      | k = str2num(get_param(gcb,'k3'));
      | alpha = str2num(get_param(gcb,'alpha3'));
      | B = str2num(get_param(gcb,'B3'));
      | Esc = str2num(get_param(gcb,'Esc3'));
      | Tins = str2num(get_param(gcb,'Tins3'));
      | I = [1.1:0.1:Esc];
      | I1=[Esc,Esc:0.1:30];
      | y=((k./((I.^alpha)-1))+B)*TMS;
      | Tin=[((k./((Esc.^alpha)-1))+B)*TMS,ones(1,length(I1)-1)*Tins];
      | loglog(I,y,'m');
      | hold on
      | loglog(I1,Tin,'m');
      | set(gcf, 'Position', [200 150 300 500]);
      | switch(get_param(gcb,'TCpopup3'))
      |     case 'IEC Standard Inverse'
      |         title('IEC Standard Inverse');
      |     case 'IEC Very Inverse'
      |         title('IEC Very Inverse');
      |     case 'IEC Long Time Inverse'
      |         title('IEC Long Time Inverse');
      |     case 'IEC Extremely Inverse'
      |         title('IEC Extremely Inverse');
      |      case 'IEC Ultra Inverse'
      |         title('IEC Ultra Inverse');
      |     case 'IEEE Moderately Inverse'
      |         title('IEEE Moderately Inverse');
      |     case 'IEEE Very Inverse'
      |         title('IEEE Very Inverse');
      |     case 'IEEE Extremely Inverse'
      |         title('IEEE Extremely Inverse');
      | end
      | ymax=10^ceil(log10(max(y)));
      | set(gca, 'XTick',[1:10 20]);
      | set(gca, 'YTick',[0 ymax/1000 ymax/500 ymax/200 ymax/100 ymax/50 ymax/20 ymax/10 ymax/5 ymax/2 ymax]);
      | xlim([0.9 30]);
      | ylim([0.01 ymax]);
      | xlabel(['Corriente multiplicada por Ipick-up(' num2str(PS*Vp) 'A)']);
      | ylabel('Tiempo de Operacion (Seg)');
      | grid on;
      | set(gca, 'color',[0.9608 0.9608 0.937]);
      | set(gca, 'gridcolor',[0 0.6902 0.3137]);
      mask Callback Esc3:
      | % Plotting IDMT Curve
      | clf('reset')
      | TMS = str2num(get_param(gcb,'TMS3'));
      | Vp = str2num(get_param(gcb,'Vp'));
      | PS=str2num(get_param(gcb,'PS3'));
      | k = str2num(get_param(gcb,'k3'));
      | alpha = str2num(get_param(gcb,'alpha3'));
      | B = str2num(get_param(gcb,'B3'));
      | Esc = str2num(get_param(gcb,'Esc3'));
      | Tins = str2num(get_param(gcb,'Tins3'));
      | I = [1.1:0.1:Esc];
      | I1=[Esc,Esc:0.1:30];
      | y=((k./((I.^alpha)-1))+B)*TMS;
      | Tin=[((k./((Esc.^alpha)-1))+B)*TMS,ones(1,length(I1)-1)*Tins];
      | loglog(I,y,'m');
      | hold on
      | loglog(I1,Tin,'m');
      | set(gcf, 'Position', [200 150 300 500]);
      | switch(get_param(gcb,'TCpopup3'))
      |     case 'IEC Standard Inverse'
      |         title('IEC Standard Inverse');
      |     case 'IEC Very Inverse'
      |         title('IEC Very Inverse');
      |     case 'IEC Long Time Inverse'
      |         title('IEC Long Time Inverse');
      |     case 'IEC Extremely Inverse'
      |         title('IEC Extremely Inverse');
      |      case 'IEC Ultra Inverse'
      |         title('IEC Ultra Inverse');
      |     case 'IEEE Moderately Inverse'
      |         title('IEEE Moderately Inverse');
      |     case 'IEEE Very Inverse'
      |         title('IEEE Very Inverse');
      |     case 'IEEE Extremely Inverse'
      |         title('IEEE Extremely Inverse');
      | end
      | ymax=10^ceil(log10(max(y)));
      | set(gca, 'XTick',[1:10 20]);
      | set(gca, 'YTick',[0 ymax/1000 ymax/500 ymax/200 ymax/100 ymax/50 ymax/20 ymax/10 ymax/5 ymax/2 ymax]);
      | xlim([0.9 30]);
      | ylim([0.01 ymax]);
      | xlabel(['Corriente multiplicada por Ipick-up(' num2str(PS*Vp) 'A)']);
      | ylabel('Tiempo de Operacion (Seg)');
      | grid on;
      | set(gca, 'color',[0.9608 0.9608 0.937]);
      | set(gca, 'gridcolor',[0 0.6902 0.3137]);
      mask DialogControl Container6 Prompt: Protecciones
      mask DialogControl Container8 Prompt: Topologia 1
      mask DialogControl Container9 Prompt: Proteccion 51
      mask DialogControl Container10 Prompt: Proteccion 50
      mask DialogControl Container8_copy Prompt: Topologia 2
      mask DialogControl Container9_copy Prompt: Proteccion 51
      mask DialogControl Container10_copy Prompt: Proteccion 50
      mask DialogControl Container8_copy_copy Prompt: Topologia 3
      mask DialogControl Container9_copy_copy Prompt: Proteccion 51
      mask DialogControl Container10_copy_copy Prompt: Proteccion 50
      mask DialogControl Container17 Prompt: Caracteristicas Trafo Corriente
      mask Display:
      | port_label('input',1,'D');
      | port_label('input',2,'I');
      | port_label('output',1,'S');
      | text(0.62, 0.5,'50', 'horizontalAlignment', 'center');
      | text(0.62, 0.3,'51', 'horizontalAlignment', 'center');
      | plot([0.08:0.01:0.32]+0.4,[0:0.01:0.24]*0+0.40);
      | plot(0.25*sin([0:pi/20:2*pi])+0.6,0.25*cos([0:pi/20:2*pi])+0.4);
      | %Linea Salida
      | plot([0.85:0.01:1],[0:0.01:0.15]*0+0.4);
      | %Linea Corriente
      | plot([0.2:0.01:0.35],[0:0.01:0.15]*0+0.4);
      | plot([0.1:0.01:0.2],[0:0.01:0.1]*0+0.15);
      | plot([0.1:0.01:0.35]*0+0.2,[0:0.01:0.25]+0.15);
      | %Linea tension
      | plot([0.15:0.01:0.6],[0:0.01:0.45]*0+0.7);
      | plot([0:0.01:0.05]*0+0.6,[0:0.01:0.05]+0.65);
  Subsystem : libreria_medidores2/Subsystem  SystemSampleTime=-1
  Subsystem1 : Subsystem  mask{tcpopup=IEC Standard Inverse, k=0.14, alpha=0.02, B=0, PS1=1.580, TMS1=0.050, Tins=0.098, Esc=10, Vp=150, Vs=5, F=60}
      mask prompts: tcpopup "Disparo"; PS1 "Plug Setting (PS)/Low-set(I>)"; TMS1 "Multiplicador Tiempo"; Esc "Escala"; Vp "Primario CT"; Vs "Secundario CT"; F "Frecuencia"
      mask TypeOptions tcpopup: IEC Standard Inverse | IEC Very Inverse | IEC Long Time Inverse | IEC Extremely Inverse | IEC Ultra Inverse | IEEE Moderately Inverse | IEEE Very Inverse | IEEE Extremely Inverse
      mask Callback tcpopup:
      | switch(get_param(gcb,'tcpopup'))
      |     case 'IEC Standard Inverse'
      |         set_param(gcb,'k','0.14');
      |         set_param(gcb,'alpha','0.02');
      |         set_param(gcb,'B','0');
      |     case 'IEC Very Inverse'
      |         set_param(gcb,'k','13.5');
      |         set_param(gcb,'alpha','1');
      |         set_param(gcb,'B','0');
      |     case 'IEC Long Time Inverse'
      |         set_param(gcb,'k','120');
      |         set_param(gcb,'alpha','1');
      |         set_param(gcb,'B','0');
      |     case 'IEC Extremely Inverse'
      |         set_param(gcb,'k','80');
      |         set_param(gcb,'alpha','2');
      |         set_param(gcb,'B','0');
      |     case 'IEC Ultra Inverse'
      |         set_param(gcb,'k','315.2');
      |         set_param(gcb,'alpha','2.5');
      |         set_param(gcb,'B','0');
      |     case 'IEEE Moderately Inverse'
      |         set_param(gcb,'k','0.0515');
      |         set_param(gcb,'alpha','0.02');
      |         set_param(gcb,'B','0.114');
      |     case 'IEEE Very Inverse'
      |         set_param(gcb,'k','19.61');
      |         set_param(gcb,'alpha','2');
      |         set_param(gcb,'B','0.491');
      |     case 'IEEE Extremely Inverse'
      |         set_param(gcb,'k','28.2');
      |         set_param(gcb,'alpha','2');
      |         set_param(gcb,'B','0.1217');
      | end
      mask DialogControl Container4 Prompt: Parametros Relee
      mask DialogControl Container13 Prompt: Proteccion 50
      mask DialogControl Container14 Prompt: Proteccion 51
      mask DialogControl Plotearcurva Prompt: Curva
      mask DialogControl Plotearcurva Callback:
      | % Plotting IDMT Curve
      | close
      | TMS = str2num(get_param(gcb,'TMS1'));
      | Vp = str2num(get_param(gcb,'Vp'));
      | PS=str2num(get_param(gcb,'PS1'));
      | k = str2num(get_param(gcb,'k'));
      | alpha = str2num(get_param(gcb,'alpha'));
      | B = str2num(get_param(gcb,'B'));
      | Esc = str2num(get_param(gcb,'Esc'));
      | Tins = str2num(get_param(gcb,'Tins'));
      | I = [1.1:0.1:Esc];
      | I1=[Esc,Esc:0.1:30]
      | y=((k./((I.^alpha)-1))+B)*TMS;
      | Tin=[((k./((Esc.^alpha)-1))+B)*TMS,ones(1,length(I1)-1)*Tins];
      | loglog(I,y,'b');
      | hold on
      | loglog(I1,Tin,'b');
      | set(gcf, 'Position', [200 150 300 500]);
      | switch(get_param(gcb,'tcpopup'))
      |     case 'IEC Standard Inverse'
      |         title('IEC Standard Inverse');
      |     case 'IEC Very Inverse'
      |         title('IEC Very Inverse');
      |     case 'IEC Long Time Inverse'
      |         title('IEC Long Time Inverse');
      |     case 'IEC Extremely Inverse'
      |         title('IEC Extremely Inverse');
      |      case 'IEC Ultra Inverse'
      |         title('IEC Ultra Inverse');
      |     case 'IEEE Moderately Inverse'
      |         title('IEEE Moderately Inverse');
      |     case 'IEEE Very Inverse'
      |         title('IEEE Very Inverse');
      |     case 'IEEE Extremely Inverse'
      |         title('IEEE Extremely Inverse');
      | end
      | ymax=10^ceil(log10(max(y)));
      | set(gca, 'XTick',[1:10 20]);
      | set(gca, 'YTick',[0 ymax/1000 ymax/500 ymax/200 ymax/100 ymax/50 ymax/20 ymax/10 ymax/5 ymax/2 ymax]);
      | xlim([0.9 30]);
      | ylim([0.01 ymax]);
      | xlabel(['Corriente multiplicada por Ipick-up(' num2str(PS*Vp) 'A)']);
      | ylabel('Operating Time (sec)');
      | grid on;
      mask DialogControl Container10 Prompt: Caracteristicas Trafo Corriente
      mask Display: disp('(50/51)');
  Subsystem10 : Subsystem  mask{tcpopup=IEC Standard Inverse, k=0.14, alpha=0.02, B=0, PS1=1.25, TMS1=0.21, Tins=0.37, Esc=57, Vp=50, Vs=5, F=60}
      mask prompts: tcpopup "Disparo"; PS1 "Plug Setting (PS)/Low-set(I>)"; TMS1 "Multiplicador Tiempo"; Esc "Escala"; Vp "Primario CT"; Vs "Secundario CT"; F "Frecuencia"
      mask TypeOptions tcpopup: IEC Standard Inverse | IEC Very Inverse | IEC Long Time Inverse | IEC Extremely Inverse | IEC Ultra Inverse | IEEE Moderately Inverse | IEEE Very Inverse | IEEE Extremely Inverse
      mask Callback tcpopup:
      | switch(get_param(gcb,'tcpopup'))
      |     case 'IEC Standard Inverse'
      |         set_param(gcb,'k','0.14');
      |         set_param(gcb,'alpha','0.02');
      |         set_param(gcb,'B','0');
      |     case 'IEC Very Inverse'
      |         set_param(gcb,'k','13.5');
      |         set_param(gcb,'alpha','1');
      |         set_param(gcb,'B','0');
      |     case 'IEC Long Time Inverse'
      |         set_param(gcb,'k','120');
      |         set_param(gcb,'alpha','1');
      |         set_param(gcb,'B','0');
      |     case 'IEC Extremely Inverse'
      |         set_param(gcb,'k','80');
      |         set_param(gcb,'alpha','2');
      |         set_param(gcb,'B','0');
      |     case 'IEC Ultra Inverse'
      |         set_param(gcb,'k','315.2');
      |         set_param(gcb,'alpha','2.5');
      |         set_param(gcb,'B','0');
      |     case 'IEEE Moderately Inverse'
      |         set_param(gcb,'k','0.0515');
      |         set_param(gcb,'alpha','0.02');
      |         set_param(gcb,'B','0.114');
      |     case 'IEEE Very Inverse'
      |         set_param(gcb,'k','19.61');
      |         set_param(gcb,'alpha','2');
      |         set_param(gcb,'B','0.491');
      |     case 'IEEE Extremely Inverse'
      |         set_param(gcb,'k','28.2');
      |         set_param(gcb,'alpha','2');
      |         set_param(gcb,'B','0.1217');
      | end
      mask DialogControl Container4 Prompt: Parametros Relee
      mask DialogControl Container13 Prompt: Proteccion 50
      mask DialogControl Container14 Prompt: Proteccion 51
      mask DialogControl Plotearcurva Prompt: Curva
      mask DialogControl Plotearcurva Callback:
      | % Plotting IDMT Curve
      | close
      | TMS = str2num(get_param(gcb,'TMS1'));
      | Vp = str2num(get_param(gcb,'Vp'));
      | PS=str2num(get_param(gcb,'PS1'));
      | k = str2num(get_param(gcb,'k'));
      | alpha = str2num(get_param(gcb,'alpha'));
      | B = str2num(get_param(gcb,'B'));
      | Esc = str2num(get_param(gcb,'Esc'));
      | Tins = str2num(get_param(gcb,'Tins'));
      | I = [1.1:0.1:Esc];
      | I1=[Esc,Esc:0.1:30]
      | y=((k./((I.^alpha)-1))+B)*TMS;
      | Tin=[((k./((Esc.^alpha)-1))+B)*TMS,ones(1,length(I1)-1)*Tins];
      | loglog(I,y,'b');
      | hold on
      | loglog(I1,Tin,'b');
      | set(gcf, 'Position', [200 150 300 500]);
      | switch(get_param(gcb,'tcpopup'))
      |     case 'IEC Standard Inverse'
      |         title('IEC Standard Inverse');
      |     case 'IEC Very Inverse'
      |         title('IEC Very Inverse');
      |     case 'IEC Long Time Inverse'
      |         title('IEC Long Time Inverse');
      |     case 'IEC Extremely Inverse'
      |         title('IEC Extremely Inverse');
      |      case 'IEC Ultra Inverse'
      |         title('IEC Ultra Inverse');
      |     case 'IEEE Moderately Inverse'
      |         title('IEEE Moderately Inverse');
      |     case 'IEEE Very Inverse'
      |         title('IEEE Very Inverse');
      |     case 'IEEE Extremely Inverse'
      |         title('IEEE Extremely Inverse');
      | end
      | ymax=10^ceil(log10(max(y)));
      | set(gca, 'XTick',[1:10 20]);
      | set(gca, 'YTick',[0 ymax/1000 ymax/500 ymax/200 ymax/100 ymax/50 ymax/20 ymax/10 ymax/5 ymax/2 ymax]);
      | xlim([0.9 30]);
      | ylim([0.01 ymax]);
      | xlabel(['Corriente multiplicada por Ipick-up(' num2str(PS*Vp) 'A)']);
      | ylabel('Operating Time (sec)');
      | grid on;
      mask DialogControl Container10 Prompt: Caracteristicas Trafo Corriente
      mask Display: disp('(50/51)');
  Subsystem3 : Subsystem  mask{tcpopup=IEC Standard Inverse, k=0.14, alpha=0.02, B=0, PS1=1, TMS1=0.34, Tins=0.758, Esc=21, Vp=300, Vs=5, F=60}
      mask prompts: tcpopup "Disparo"; PS1 "Plug Setting (PS)/Low-set(I>)"; TMS1 "Multiplicador Tiempo"; Esc "Escala"; Vp "Primario CT"; Vs "Secundario CT"; F "Frecuencia"
      mask TypeOptions tcpopup: IEC Standard Inverse | IEC Very Inverse | IEC Long Time Inverse | IEC Extremely Inverse | IEC Ultra Inverse | IEEE Moderately Inverse | IEEE Very Inverse | IEEE Extremely Inverse
      mask Callback tcpopup:
      | switch(get_param(gcb,'tcpopup'))
      |     case 'IEC Standard Inverse'
      |         set_param(gcb,'k','0.14');
      |         set_param(gcb,'alpha','0.02');
      |         set_param(gcb,'B','0');
      |     case 'IEC Very Inverse'
      |         set_param(gcb,'k','13.5');
      |         set_param(gcb,'alpha','1');
      |         set_param(gcb,'B','0');
      |     case 'IEC Long Time Inverse'
      |         set_param(gcb,'k','120');
      |         set_param(gcb,'alpha','1');
      |         set_param(gcb,'B','0');
      |     case 'IEC Extremely Inverse'
      |         set_param(gcb,'k','80');
      |         set_param(gcb,'alpha','2');
      |         set_param(gcb,'B','0');
      |     case 'IEC Ultra Inverse'
      |         set_param(gcb,'k','315.2');
      |         set_param(gcb,'alpha','2.5');
